simulink model "PreCondition"  (R2018b)
settings: Solver=FixedStepDiscrete  StartTime=0.0  StopTime=10.0  FixedStep=0.01  RelTol=1e-3
undefined symbols (not defined in the file or in its folder): EnergyMgLdShdRq1, HMI_2L_StMd10_Config_Val, HMI_2L_StMd11_Config_Val, HMI_2L_StMd12_Config_Val, HMI_2L_StMd13_Config_Val, HMI_2L_StMd14_Config_Val, HMI_2L_StMd15_Config_Val, HMI_2L_StMd16_Config_Val, HMI_2L_StMd17_Config_Val, HMI_2L_StMd18_Config_Val, HMI_2L_StMd19_Config_Val, HMI_2L_StMd1_Config_Val, HMI_2L_StMd20_Config_Val, HMI_2L_StMd21_Config_Val, HMI_2L_StMd22_Config_Val, HMI_2L_StMd23_Config_Val, HMI_2L_StMd24_Config_Val, HMI_2L_StMd25_Config_Val, HMI_2L_StMd26_Config_Val, HMI_2L_StMd27_Config_Val, HMI_2L_StMd28_Config_Val, HMI_2L_StMd29_Config_Val, HMI_2L_StMd2_Config_Val, HMI_2L_StMd30_Config_Val, HMI_2L_StMd31_Config_Val, HMI_2L_StMd32_Config_Val, HMI_2L_StMd3_Config_Val, HMI_2L_StMd4_Config_Val, HMI_2L_StMd5_Config_Val, HMI_2L_StMd6_Config_Val, HMI_2L_StMd7_Config_Val, HMI_2L_StMd8_Config_Val, HMI_2L_StMd9_Config_Val, HMI_2R_StMd10_Config_Val, HMI_2R_StMd11_Config_Val, HMI_2R_StMd12_Config_Val, HMI_2R_StMd13_Config_Val, HMI_2R_StMd14_Config_Val, HMI_2R_StMd15_Config_Val, HMI_2R_StMd16_Config_Val, HMI_2R_StMd17_Config_Val, HMI_2R_StMd18_Config_Val, HMI_2R_StMd19_Config_Val, HMI_2R_StMd1_Config_Val, HMI_2R_StMd20_Config_Val, HMI_2R_StMd21_Config_Val, HMI_2R_StMd22_Config_Val, HMI_2R_StMd23_Config_Val, HMI_2R_StMd24_Config_Val, HMI_2R_StMd25_Config_Val, HMI_2R_StMd26_Config_Val, HMI_2R_StMd27_Config_Val, HMI_2R_StMd28_Config_Val, HMI_2R_StMd29_Config_Val, HMI_2R_StMd2_Config_Val, HMI_2R_StMd30_Config_Val, HMI_2R_StMd31_Config_Val, HMI_2R_StMd32_Config_Val, HMI_2R_StMd3_Config_Val, HMI_2R_StMd4_Config_Val ... (+94)
(part 3 of 6)

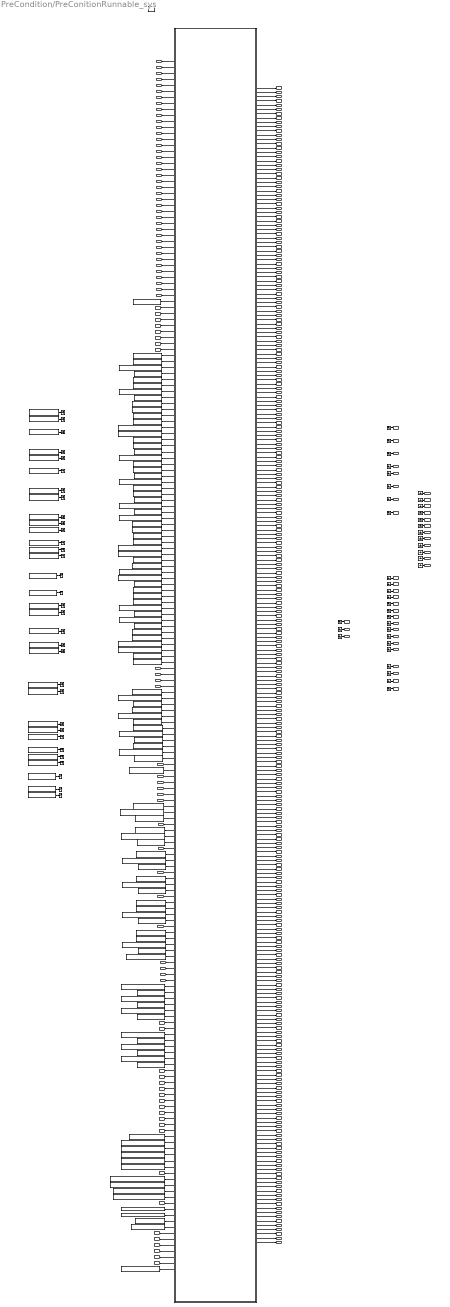
== system PreCondition/PreConitionRunnable_sys ==
  AbgDplyBckp_Val_read : Inport
  AbgDplyBckpV_Val_read : Inport  Port=2
  AcsEntryPosLrnd_Val_read : Inport  Port=3
  DrvStPosRclRspStat_Val_read : Inport  Port=4
  EnergyMgLdShdRq_Val_read : Inport  Port=5
  FamilyLtPosLrnd_Val_read : Inport  Port=6
  FamilyRtPosLrnd_Val_read : Inport  Port=7
  IfVeSMSeStNumConfig_Val_read : Inport  Port=8
  IntimacyLPosLrnd_Val_read : Inport  Port=9
  IntimacyRPosLrnd_Val_read : Inport  Port=10
  Is2LStSwAct_Val_read : Inport  Port=11
  Is2RStSwAct_Val_read : Inport  Port=12
  Is3LStSwAct_Val_read : Inport  Port=13
  Is3RStSwAct_Val_read : Inport  Port=14
  IsDrvStSwAct_Val_read : Inport  Port=15
  IsPasStSwAct_Val_read : Inport  Port=16
  LgrstCloseLtPosLrnd_Val_read : Inport  Port=17
  LgrstCloseRtPosLrnd_Val_read : Inport  Port=18
  LgrstOpenLtPosLrnd_Val_read : Inport  Port=19
  LgrstOpenRtPosLrnd_Val_read : Inport  Port=20
  LugLtPosLrnd_Val_read : Inport  Port=21
  LugRtPosLrnd_Val_read : Inport  Port=22
  LyingLtPosLrnd_Val_read : Inport  Port=23
  LyingRtPosLrnd_Val_read : Inport  Port=24
  MmryRclImpctDisRq_Val_read : Inport  Port=25
  AcsExitPosLrnd_Val_read : Inport  Port=26
  PassStPosRclRspStat_Val_read : Inport  Port=27
  VIPLtPosLrnd_Val_read : Inport  Port=28
  SecRwLtStChldLkReq_Val_read : Inport  Port=29
  SecRwLtStPosRclRspStat_Val_read : Inport  Port=30
  VIPRtPosLrnd_Val_read : Inport  Port=31
  SecRwRtStChldLkReq_Val_read : Inport  Port=32
  SecRwRtStPosRclRspStat_Val_read : Inport  Port=33
  SysPwrMd_Val_read : Inport  Port=34
  SysPwrMdV_Val_read : Inport  Port=35
  ThdRwCtStOccStatMSMSrc_Val_read : Inport  Port=36
  RcvyLtPosLrnd_Val_read : Inport  Port=37
  ThdRwLtStOccStatMSMSrc_Val_read : Inport  Port=38
  ThdRwLtStPosRclRspStat_Val_read : Inport  Port=39
  RcvyRtPosLrnd_Val_read : Inport  Port=40
  ThdRwRtStOccStatMSMSrc_Val_read : Inport  Port=41
  ThdRwRtStPosRclRspStat_Val_read : Inport  Port=42
  VehMovState_Val_read : Inport  Port=43
  VehSpdAvgDrvn_Val_read : Inport  Port=44
  VehSpdAvgDrvnV_Val_read : Inport  Port=45
  VeSignalLost2R_463_2L_Val_read : Inport  Port=46
  VeSignalLost3L_468_2L_Val_read : Inport  Port=47
  VeSignalLost3R_46C_2L_Val_read : Inport  Port=48
  VeSignalLostCODR_470_2L_Val_read : Inport  Port=49
  VeSignalLostDR_213_2L_Val_read : Inport  Port=50
  VeSignalLostFireWall_1D2_2L_Val_read : Inport  Port=51
  VeSignalLostSDM_195_2L_Val_read : Inport  Port=52
  VoltSts_Val_read : Inport  Port=53
  SecRwLtStFrwdBkwdPos_Val_read : Inport  Port=54
  SecRwLtStFrwdBkwdPosV_Val_read : Inport  Port=55
  SecRwRtStFrwdBkwdPos_Val_read : Inport  Port=56
  SecRwRtStFrwdBkwdPosV_Val_read : Inport  Port=57
  AcsEntry4s2LPosLrnd_Val_read : Inport  Port=58
  AcsEntry4s2RPosLrnd_Val_read : Inport  Port=59
  AcsEntryAll4sBwdPosLrnd_Val_read : Inport  Port=60
  AcsEntryAll4sFwdPosLrnd_Val_read : Inport  Port=61
  AcsExit4s2LPosLrnd_Val_read : Inport  Port=62
  AcsExit4s2RPosLrnd_Val_read : Inport  Port=63
  IfVeSMSbPassReclinerPosLrnd_Val_read : Inport  Port=64
  IfVeSMSbunfold3LPosLrnd_Val_read : Inport  Port=65
  IfVeSMSbunfold3RPosLrnd_Val_read : Inport  Port=66
  NotCoDrvStOccStatBDFSrc_Val_read : Inport  Port=67
  IfVeSMSbVIPLtOutPosLrnd_Val_read : Inport  Port=68
  IfVeSMSbVIPRtOutPosLrnd_Val_read : Inport  Port=69
  IfVeSMSuThdRwLtStCshnFldUpwdDnwdPos_Val_read : Inport  Port=70
  IfVeSMSuThdRwLtStCshnFldUpwdDnwdPosV_Val_read : Inport  Port=71
  IfVeSMSuThdRwRtStCshnFldUpwdDnwdPos_Val_read : Inport  Port=72
  IfVeSMSuThdRwRtStCshnFldUpwdDnwdPosV_Val_read : Inport  Port=73
  ThdRwLtStChldLkReq_Val_read : Inport  Port=74
  NotSecRowLeStOccStatBDFSrc_Val_read : Inport  Port=75
  NotSecRowRtStOccStatBDFSrc_Val_read : Inport  Port=76
  IfVeSMSbSecRwLtStBkReclnUpwdDnwdPosV_Val_read : Inport  Port=77
  IfVeSMSbSecRwRtStBkReclnUpwdDnwdPosV_Val_read : Inport  Port=78
  IfVeSMSuSecRwLtStBkReclnUpwdDnwdPos_Val_read : Inport  Port=79
  IfVeSMSuSecRwRtStBkReclnUpwdDnwdPos_Val_read : Inport  Port=80
  IfVeSMSbPasReclinerPosAvail_Val_read : Inport  Port=81
  WholeVehMemPosLrnd_Val_read : Inport  Port=82
  Md61PassStBkReclnTrgtPos_Val_read : Inport  Port=83
  Md61ThdRwLtStCshnFldUpwdDnwdTrgtPos_Val_read : Inport  Port=84
  Md61ThdRwRtStCshnFldUpwdDnwdTrgtPos_Val_read : Inport  Port=85
  Md62PassStBkReclnTrgtPos_Val_read : Inport  Port=86
  Md62ThdRwLtStCshnFldUpwdDnwdTrgtPos_Val_read : Inport  Port=87
  Md62ThdRwRtStCshnFldUpwdDnwdTrgtPos_Val_read : Inport  Port=88
  function : TriggerPort  TriggerType=function-call  VariantControl=(inherit)  SampleTimeType=periodic  SampleTime=-1
  Ground_{36,40,43,47,55,57,60,62,64,66..67,69,71,73,83..94,99..110,120} (39 alike) : Ground
  PA_HMI_2L_StMd10_Config_Val : Constant  Value=HMI_2L_StMd10_Config_Val
  PA_HMI_2L_StMd11_Config_Val : Constant  Value=HMI_2L_StMd11_Config_Val
  PA_HMI_2L_StMd12_Config_Val : Constant  Value=HMI_2L_StMd12_Config_Val
  PA_HMI_2L_StMd13_Config_Val : Constant  Value=HMI_2L_StMd13_Config_Val
  PA_HMI_2L_StMd14_Config_Val : Constant  Value=HMI_2L_StMd14_Config_Val
  PA_HMI_2L_StMd15_Config_Val : Constant  Value=HMI_2L_StMd15_Config_Val
  PA_HMI_2L_StMd16_Config_Val : Constant  Value=HMI_2L_StMd16_Config_Val
  PA_HMI_2L_StMd17_Config_Val : Constant  Value=HMI_2L_StMd17_Config_Val
  PA_HMI_2L_StMd18_Config_Val : Constant  Value=HMI_2L_StMd18_Config_Val
  PA_HMI_2L_StMd19_Config_Val : Constant  Value=HMI_2L_StMd19_Config_Val
  PA_HMI_2L_StMd1_Config_Val : Constant  Value=HMI_2L_StMd1_Config_Val
  PA_HMI_2L_StMd20_Config_Val : Constant  Value=HMI_2L_StMd20_Config_Val
  PA_HMI_2L_StMd21_Config_Val : Constant  Value=HMI_2L_StMd21_Config_Val
  PA_HMI_2L_StMd22_Config_Val : Constant  Value=HMI_2L_StMd22_Config_Val
  PA_HMI_2L_StMd23_Config_Val : Constant  Value=HMI_2L_StMd23_Config_Val
  PA_HMI_2L_StMd24_Config_Val : Constant  Value=HMI_2L_StMd24_Config_Val
  PA_HMI_2L_StMd25_Config_Val : Constant  Value=HMI_2L_StMd25_Config_Val
  PA_HMI_2L_StMd26_Config_Val : Constant  Value=HMI_2L_StMd26_Config_Val
  PA_HMI_2L_StMd27_Config_Val : Constant  Value=HMI_2L_StMd27_Config_Val
  PA_HMI_2L_StMd28_Config_Val : Constant  Value=HMI_2L_StMd28_Config_Val
  PA_HMI_2L_StMd29_Config_Val : Constant  Value=HMI_2L_StMd29_Config_Val
  PA_HMI_2L_StMd2_Config_Val : Constant  Value=HMI_2L_StMd2_Config_Val
  PA_HMI_2L_StMd30_Config_Val : Constant  Value=HMI_2L_StMd30_Config_Val
  PA_HMI_2L_StMd31_Config_Val : Constant  Value=HMI_2L_StMd31_Config_Val
  PA_HMI_2L_StMd32_Config_Val : Constant  Value=HMI_2L_StMd32_Config_Val
  PA_HMI_2L_StMd3_Config_Val : Constant  Value=HMI_2L_StMd3_Config_Val
  PA_HMI_2L_StMd4_Config_Val : Constant  Value=HMI_2L_StMd4_Config_Val
  PA_HMI_2L_StMd5_Config_Val : Constant  Value=HMI_2L_StMd5_Config_Val
  PA_HMI_2L_StMd6_Config_Val : Constant  Value=HMI_2L_StMd6_Config_Val
  PA_HMI_2L_StMd7_Config_Val : Constant  Value=HMI_2L_StMd7_Config_Val
  PA_HMI_2L_StMd8_Config_Val : Constant  Value=HMI_2L_StMd8_Config_Val
  PA_HMI_2L_StMd9_Config_Val : Constant  Value=HMI_2L_StMd9_Config_Val
  PA_HMI_2R_StMd10_Config_Val : Constant  Value=HMI_2R_StMd10_Config_Val
  PA_HMI_2R_StMd11_Config_Val : Constant  Value=HMI_2R_StMd11_Config_Val
  PA_HMI_2R_StMd12_Config_Val : Constant  Value=HMI_2R_StMd12_Config_Val
  PA_HMI_2R_StMd13_Config_Val : Constant  Value=HMI_2R_StMd13_Config_Val
  PA_HMI_2R_StMd14_Config_Val : Constant  Value=HMI_2R_StMd14_Config_Val
  PA_HMI_2R_StMd15_Config_Val : Constant  Value=HMI_2R_StMd15_Config_Val
  PA_HMI_2R_StMd16_Config_Val : Constant  Value=HMI_2R_StMd16_Config_Val
  PA_HMI_2R_StMd17_Config_Val : Constant  Value=HMI_2R_StMd17_Config_Val
  PA_HMI_2R_StMd18_Config_Val : Constant  Value=HMI_2R_StMd18_Config_Val
  PA_HMI_2R_StMd19_Config_Val : Constant  Value=HMI_2R_StMd19_Config_Val
  PA_HMI_2R_StMd1_Config_Val : Constant  Value=HMI_2R_StMd1_Config_Val
  PA_HMI_2R_StMd20_Config_Val : Constant  Value=HMI_2R_StMd20_Config_Val
  PA_HMI_2R_StMd21_Config_Val : Constant  Value=HMI_2R_StMd21_Config_Val
  PA_HMI_2R_StMd22_Config_Val : Constant  Value=HMI_2R_StMd22_Config_Val
  PA_HMI_2R_StMd23_Config_Val : Constant  Value=HMI_2R_StMd23_Config_Val
  PA_HMI_2R_StMd24_Config_Val : Constant  Value=HMI_2R_StMd24_Config_Val
  PA_HMI_2R_StMd25_Config_Val : Constant  Value=HMI_2R_StMd25_Config_Val
  PA_HMI_2R_StMd26_Config_Val : Constant  Value=HMI_2R_StMd26_Config_Val
  PA_HMI_2R_StMd27_Config_Val : Constant  Value=HMI_2R_StMd27_Config_Val
  PA_HMI_2R_StMd28_Config_Val : Constant  Value=HMI_2R_StMd28_Config_Val
  PA_HMI_2R_StMd29_Config_Val : Constant  Value=HMI_2R_StMd29_Config_Val
  PA_HMI_2R_StMd2_Config_Val : Constant  Value=HMI_2R_StMd2_Config_Val
  PA_HMI_2R_StMd30_Config_Val : Constant  Value=HMI_2R_StMd30_Config_Val
  PA_HMI_2R_StMd31_Config_Val : Constant  Value=HMI_2R_StMd31_Config_Val
  PA_HMI_2R_StMd32_Config_Val : Constant  Value=HMI_2R_StMd32_Config_Val
  PA_HMI_2R_StMd3_Config_Val : Constant  Value=HMI_2R_StMd3_Config_Val
  PA_HMI_2R_StMd4_Config_Val : Constant  Value=HMI_2R_StMd4_Config_Val
  PA_HMI_2R_StMd5_Config_Val : Constant  Value=HMI_2R_StMd5_Config_Val
  PA_HMI_2R_StMd6_Config_Val : Constant  Value=HMI_2R_StMd6_Config_Val
  PA_HMI_2R_StMd7_Config_Val : Constant  Value=HMI_2R_StMd7_Config_Val
  PA_HMI_2R_StMd8_Config_Val : Constant  Value=HMI_2R_StMd8_Config_Val
  PA_HMI_2R_StMd9_Config_Val : Constant  Value=HMI_2R_StMd9_Config_Val
  PA_IfKeSMSbSeatMovFrwdBkwdEnable_Val : Constant  Value=IfKeSMSbSeatMovFrwdBkwdEnable_Val
  PA_KeSMSLegrstDisFwdBkwdPos_Val : Constant  Value=KeSMSLegrstDisFwdBkwdPos_Val
  PA_KeSMSbRoofSWEnable_Val : Constant  Value=KeSMSbRoofSWEnable_Val
  PA_KeSMSuSecRwStBackPosDelta_Val : Constant  Value=KeSMSuSecRwStBackPosDelta_Val
  PA_KeSMSuThrdRwCushFoldPosDelta_Val : Constant  Value=KeSMSuThrdRwCushFoldPosDelta_Val
  PA_KeSMSuThrdRwCushFoldPosThreshold_Val : Constant  Value=KeSMSuThrdRwCushFoldPosThreshold_Val
  PA_KeSMSwAcsMd32SecRwLtStBkReclnUpwdDnwdPos1_Val : Constant  Value=KeSMSwAcsMd32SecRwLtStBkReclnUpwdDnwdPos1_Val
  PA_KeSMSwAcsMd53SecRwRtStBkReclnUpwdDnwdPos1_Val : Constant  Value=KeSMSwAcsMd53SecRwRtStBkReclnUpwdDnwdPos1_Val
  PA_KeSMSwAcsMd8SecRwLtStBkReclnUpwdDnwdPos_Val : Constant  Value=KeSMSwAcsMd8SecRwLtStBkReclnUpwdDnwdPos_Val
  PA_KeSMSwAcsMd9SecRwRtStBkReclnUpwdDnwdPos_Val : Constant  Value=KeSMSwAcsMd9SecRwRtStBkReclnUpwdDnwdPos_Val
  PA_KeSMSwSeatBkLimitPosDelt_Val : Constant  Value=KeSMSwSeatBkLimitPosDelt_Val
  PA_KeSMSwSeatBkLimitPos_Val : Constant  Value=KeSMSwSeatBkLimitPos_Val
  PA_StPassCmprtMdCtrl_Md10_VCUConfig_Val : Constant  Value=StPassCmprtMdCtrl_Md10_VCUConfig_Val
  PA_StPassCmprtMdCtrl_Md11_VCUConfig_Val : Constant  Value=StPassCmprtMdCtrl_Md11_VCUConfig_Val
  PA_StPassCmprtMdCtrl_Md12_VCUConfig_Val : Constant  Value=StPassCmprtMdCtrl_Md12_VCUConfig_Val
  PA_StPassCmprtMdCtrl_Md13_VCUConfig_Val : Constant  Value=StPassCmprtMdCtrl_Md13_VCUConfig_Val
  PA_StPassCmprtMdCtrl_Md14_VCUConfig_Val : Constant  Value=StPassCmprtMdCtrl_Md14_VCUConfig_Val
  PA_StPassCmprtMdCtrl_Md15_VCUConfig_Val : Constant  Value=StPassCmprtMdCtrl_Md15_VCUConfig_Val
  PA_StPassCmprtMdCtrl_Md16_VCUConfig_Val : Constant  Value=StPassCmprtMdCtrl_Md16_VCUConfig_Val
  PA_StPassCmprtMdCtrl_Md17_VCUConfig_Val : Constant  Value=StPassCmprtMdCtrl_Md17_VCUConfig_Val
  PA_StPassCmprtMdCtrl_Md18_VCUConfig_Val : Constant  Value=StPassCmprtMdCtrl_Md18_VCUConfig_Val
  PA_StPassCmprtMdCtrl_Md19_VCUConfig_Val : Constant  Value=StPassCmprtMdCtrl_Md19_VCUConfig_Val
  PA_StPassCmprtMdCtrl_Md1_VCUConfig_Val : Constant  Value=StPassCmprtMdCtrl_Md1_VCUConfig_Val
  PA_StPassCmprtMdCtrl_Md20_VCUConfig_Val : Constant  Value=StPassCmprtMdCtrl_Md20_VCUConfig_Val
  PA_StPassCmprtMdCtrl_Md21_VCUConfig_Val : Constant  Value=StPassCmprtMdCtrl_Md21_VCUConfig_Val
  PA_StPassCmprtMdCtrl_Md22_VCUConfig_Val : Constant  Value=StPassCmprtMdCtrl_Md22_VCUConfig_Val
  PA_StPassCmprtMdCtrl_Md23_VCUConfig_Val : Constant  Value=StPassCmprtMdCtrl_Md23_VCUConfig_Val
  PA_StPassCmprtMdCtrl_Md24_VCUConfig_Val : Constant  Value=StPassCmprtMdCtrl_Md24_VCUConfig_Val
  PA_StPassCmprtMdCtrl_Md25_VCUConfig_Val : Constant  Value=StPassCmprtMdCtrl_Md25_VCUConfig_Val
  PA_StPassCmprtMdCtrl_Md26_VCUConfig_Val : Constant  Value=StPassCmprtMdCtrl_Md26_VCUConfig_Val
  PA_StPassCmprtMdCtrl_Md27_VCUConfig_Val : Constant  Value=StPassCmprtMdCtrl_Md27_VCUConfig_Val
  PA_StPassCmprtMdCtrl_Md28_VCUConfig_Val : Constant  Value=StPassCmprtMdCtrl_Md28_VCUConfig_Val
  PA_StPassCmprtMdCtrl_Md29_VCUConfig_Val : Constant  Value=StPassCmprtMdCtrl_Md29_VCUConfig_Val
  PA_StPassCmprtMdCtrl_Md2_VCUConfig_Val : Constant  Value=StPassCmprtMdCtrl_Md2_VCUConfig_Val
  PA_StPassCmprtMdCtrl_Md30_VCUConfig_Val : Constant  Value=StPassCmprtMdCtrl_Md30_VCUConfig_Val
  PA_StPassCmprtMdCtrl_Md31_VCUConfig_Val : Constant  Value=StPassCmprtMdCtrl_Md31_VCUConfig_Val
  PA_StPassCmprtMdCtrl_Md32_VCUConfig_Val : Constant  Value=StPassCmprtMdCtrl_Md32_VCUConfig_Val
  PA_StPassCmprtMdCtrl_Md3_VCUConfig_Val : Constant  Value=StPassCmprtMdCtrl_Md3_VCUConfig_Val
  PA_StPassCmprtMdCtrl_Md4_VCUConfig_Val : Constant  Value=StPassCmprtMdCtrl_Md4_VCUConfig_Val
  PA_StPassCmprtMdCtrl_Md53_VCUConfig_Val : Constant  Value=StPassCmprtMdCtrl_Md53_VCUConfig_Val
  PA_StPassCmprtMdCtrl_Md56_VCUConfig_Val : Constant  Value=StPassCmprtMdCtrl_Md56_VCUConfig_Val
  PA_StPassCmprtMdCtrl_Md57_VCUConfig_Val : Constant  Value=StPassCmprtMdCtrl_Md57_VCUConfig_Val
  PA_StPassCmprtMdCtrl_Md58_VCUConfig_Val : Constant  Value=StPassCmprtMdCtrl_Md58_VCUConfig_Val
  PA_StPassCmprtMdCtrl_Md5_VCUConfig_Val : Constant  Value=StPassCmprtMdCtrl_Md5_VCUConfig_Val
  PA_StPassCmprtMdCtrl_Md61_VCUConfig_Val : Constant  Value=StPassCmprtMdCtrl_Md61_VCUConfig_Val
  PA_StPassCmprtMdCtrl_Md62_VCUConfig_Val : Constant  Value=StPassCmprtMdCtrl_Md62_VCUConfig_Val
  PA_StPassCmprtMdCtrl_Md6_VCUConfig_Val : Constant  Value=StPassCmprtMdCtrl_Md6_VCUConfig_Val
  PA_StPassCmprtMdCtrl_Md7_VCUConfig_Val : Constant  Value=StPassCmprtMdCtrl_Md7_VCUConfig_Val
  PA_StPassCmprtMdCtrl_Md8_VCUConfig_Val : Constant  Value=StPassCmprtMdCtrl_Md8_VCUConfig_Val
  PA_StPassCmprtMdCtrl_Md9_VCUConfig_Val : Constant  Value=StPassCmprtMdCtrl_Md9_VCUConfig_Val
  PA_StSrv_StMd10_Config_Val : Constant  Value=StSrv_StMd10_Config_Val
  PA_StSrv_StMd11_Config_Val : Constant  Value=StSrv_StMd11_Config_Val
  PA_StSrv_StMd12_Config_Val : Constant  Value=StSrv_StMd12_Config_Val
  PA_StSrv_StMd13_Config_Val : Constant  Value=StSrv_StMd13_Config_Val
  PA_StSrv_StMd14_Config_Val : Constant  Value=StSrv_StMd14_Config_Val
  PA_StSrv_StMd15_Config_Val : Constant  Value=StSrv_StMd15_Config_Val
  PA_StSrv_StMd16_Config_Val : Constant  Value=StSrv_StMd16_Config_Val
  PA_StSrv_StMd17_Config_Val : Constant  Value=StSrv_StMd17_Config_Val
  PA_StSrv_StMd18_Config_Val : Constant  Value=StSrv_StMd18_Config_Val
  PA_StSrv_StMd19_Config_Val : Constant  Value=StSrv_StMd19_Config_Val
  PA_StSrv_StMd1_Config_Val : Constant  Value=StSrv_StMd1_Config_Val
  PA_StSrv_StMd20_Config_Val : Constant  Value=StSrv_StMd20_Config_Val
  PA_StSrv_StMd21_Config_Val : Constant  Value=StSrv_StMd21_Config_Val
  PA_StSrv_StMd22_Config_Val : Constant  Value=StSrv_StMd22_Config_Val
  PA_StSrv_StMd23_Config_Val : Constant  Value=StSrv_StMd23_Config_Val
  PA_StSrv_StMd24_Config_Val : Constant  Value=StSrv_StMd24_Config_Val
  PA_StSrv_StMd25_Config_Val : Constant  Value=StSrv_StMd25_Config_Val
  PA_StSrv_StMd26_Config_Val : Constant  Value=StSrv_StMd26_Config_Val
  PA_StSrv_StMd27_Config_Val : Constant  Value=StSrv_StMd27_Config_Val
  PA_StSrv_StMd28_Config_Val : Constant  Value=StSrv_StMd28_Config_Val
  PA_StSrv_StMd29_Config_Val : Constant  Value=StSrv_StMd29_Config_Val
  PA_StSrv_StMd2_Config_Val : Constant  Value=StSrv_StMd2_Config_Val
  PA_StSrv_StMd30_Config_Val : Constant  Value=StSrv_StMd30_Config_Val
  PA_StSrv_StMd31_Config_Val : Constant  Value=StSrv_StMd31_Config_Val
  PA_StSrv_StMd32_Config_Val : Constant  Value=StSrv_StMd32_Config_Val
  PA_StSrv_StMd3_Config_Val : Constant  Value=StSrv_StMd3_Config_Val
  PA_StSrv_StMd4_Config_Val : Constant  Value=StSrv_StMd4_Config_Val
  PA_StSrv_StMd5_Config_Val : Constant  Value=StSrv_StMd5_Config_Val
  PA_StSrv_StMd6_Config_Val : Constant  Value=StSrv_StMd6_Config_Val
  PA_StSrv_StMd7_Config_Val : Constant  Value=StSrv_StMd7_Config_Val
  PA_StSrv_StMd8_Config_Val : Constant  Value=StSrv_StMd8_Config_Val
  PA_StSrv_StMd9_Config_Val : Constant  Value=StSrv_StMd9_Config_Val
  Subsystem3 : Subsystem
  Terminator_{56..57,59,62..63,65,68..69,72..74,76..78,82,85..87,90,92..93,98..99,104..106,108..110,113,115..116} (32 alike) : Terminator
  AcsMdEntyAvl_Val_write : Outport
  AcsMdExtAvl_Val_write : Outport  Port=2
  CommCond_Val_write : Outport  Port=3
  CommExitCond_Val_write : Outport  Port=4
  CommExitCondwithSpeed_Val_write : Outport  Port=5
  DiagAbgDly_Val_write : Outport  Port=6
  DiagVehMovState_Val_write : Outport  Port=7
  DiagVehSpdAvgDrvn_Val_write : Outport  Port=8
  FamilyMdLtAvl_Val_write : Outport  Port=9
  FamilyMdRtAvl_Val_write : Outport  Port=10
  HMIMd10Avl_2L_Val_write : Outport  Port=11
  HMIMd10Avl_2R_Val_write : Outport  Port=12
  HMIMd10Cfg_2L_Val_write : Outport  Port=13
  HMIMd10Cfg_2R_Val_write : Outport  Port=14
  HMIMd11Avl_2L_Val_write : Outport  Port=15
  HMIMd11Avl_2R_Val_write : Outport  Port=16
  HMIMd11Cfg_2L_Val_write : Outport  Port=17
  HMIMd11Cfg_2R_Val_write : Outport  Port=18
  HMIMd12Avl_2L_Val_write : Outport  Port=19
  HMIMd12Avl_2R_Val_write : Outport  Port=20
  HMIMd12Cfg_2L_Val_write : Outport  Port=21
  HMIMd12Cfg_2R_Val_write : Outport  Port=22
  HMIMd13Avl_2L_Val_write : Outport  Port=23
  HMIMd13Avl_2R_Val_write : Outport  Port=24
  HMIMd13Cfg_2L_Val_write : Outport  Port=25
  HMIMd13Cfg_2R_Val_write : Outport  Port=26
  HMIMd14Avl_2L_Val_write : Outport  Port=27
  HMIMd14Avl_2R_Val_write : Outport  Port=28
  HMIMd14Cfg_2L_Val_write : Outport  Port=29
  HMIMd14Cfg_2R_Val_write : Outport  Port=30
  HMIMd15Avl_2L_Val_write : Outport  Port=31
  HMIMd15Avl_2R_Val_write : Outport  Port=32
  HMIMd15Cfg_2L_Val_write : Outport  Port=33
  HMIMd15Cfg_2R_Val_write : Outport  Port=34
  HMIMd16Avl_2L_Val_write : Outport  Port=35
  HMIMd16Avl_2R_Val_write : Outport  Port=36
      settings: EnsureOutportIsVirtual=on
  HMIMd16Cfg_2L_Val_write : Outport  Port=37
  HMIMd16Cfg_2R_Val_write : Outport  Port=38
  HMIMd17Avl_2L_Val_write : Outport  Port=39
  HMIMd17Avl_2R_Val_write : Outport  Port=40
      settings: EnsureOutportIsVirtual=on
  HMIMd17Cfg_2L_Val_write : Outport  Port=41
  HMIMd17Cfg_2R_Val_write : Outport  Port=42
  HMIMd18Avl_2L_Val_write : Outport  Port=43
      settings: EnsureOutportIsVirtual=on
  HMIMd18Avl_2R_Val_write : Outport  Port=44
  HMIMd18Cfg_2L_Val_write : Outport  Port=45
  HMIMd18Cfg_2R_Val_write : Outport  Port=46
  HMIMd19Avl_2L_Val_write : Outport  Port=47
      settings: EnsureOutportIsVirtual=on
  HMIMd19Avl_2R_Val_write : Outport  Port=48
  HMIMd19Cfg_2L_Val_write : Outport  Port=49
  HMIMd19Cfg_2R_Val_write : Outport  Port=50
  HMIMd1Avl_2L_Val_write : Outport  Port=51
  HMIMd1Avl_2R_Val_write : Outport  Port=52
  HMIMd1Cfg_2L_Val_write : Outport  Port=53
  HMIMd1Cfg_2R_Val_write : Outport  Port=54
  HMIMd20Avl_2L_Val_write : Outport  Port=55
      settings: EnsureOutportIsVirtual=on
  HMIMd20Avl_2R_Val_write : Outport  Port=56
  HMIMd20Cfg_2L_Val_write : Outport  Port=57
      settings: EnsureOutportIsVirtual=on
  HMIMd20Cfg_2R_Val_write : Outport  Port=58
  HMIMd21Avl_2L_Val_write : Outport  Port=59
  HMIMd21Avl_2R_Val_write : Outport  Port=60
      settings: EnsureOutportIsVirtual=on
  HMIMd21Cfg_2L_Val_write : Outport  Port=61
  HMIMd21Cfg_2R_Val_write : Outport  Port=62
      settings: EnsureOutportIsVirtual=on
  HMIMd22Avl_2L_Val_write : Outport  Port=63
  HMIMd22Avl_2R_Val_write : Outport  Port=64
      settings: EnsureOutportIsVirtual=on
  HMIMd22Cfg_2L_Val_write : Outport  Port=65
  HMIMd22Cfg_2R_Val_write : Outport  Port=66
      settings: EnsureOutportIsVirtual=on
  HMIMd23Avl_2L_Val_write : Outport  Port=67
      settings: EnsureOutportIsVirtual=on
  HMIMd23Avl_2R_Val_write : Outport  Port=68
  HMIMd23Cfg_2L_Val_write : Outport  Port=69
      settings: EnsureOutportIsVirtual=on
  HMIMd23Cfg_2R_Val_write : Outport  Port=70
  HMIMd24Avl_2L_Val_write : Outport  Port=71
      settings: EnsureOutportIsVirtual=on
  HMIMd24Avl_2R_Val_write : Outport  Port=72
  HMIMd24Cfg_2L_Val_write : Outport  Port=73
      settings: EnsureOutportIsVirtual=on
  HMIMd24Cfg_2R_Val_write : Outport  Port=74
  HMIMd25Avl_2L_Val_write : Outport  Port=75
  HMIMd25Avl_2R_Val_write : Outport  Port=76
  HMIMd25Cfg_2L_Val_write : Outport  Port=77
  HMIMd25Cfg_2R_Val_write : Outport  Port=78
  HMIMd26Avl_2L_Val_write : Outport  Port=79
  HMIMd26Avl_2R_Val_write : Outport  Port=80
  HMIMd26Cfg_2L_Val_write : Outport  Port=81
  HMIMd26Cfg_2R_Val_write : Outport  Port=82
  HMIMd27Avl_2L_Val_write : Outport  Port=83
      settings: EnsureOutportIsVirtual=on
  HMIMd27Avl_2R_Val_write : Outport  Port=84
      settings: EnsureOutportIsVirtual=on
  HMIMd27Cfg_2L_Val_write : Outport  Port=85
      settings: EnsureOutportIsVirtual=on
  HMIMd27Cfg_2R_Val_write : Outport  Port=86
      settings: EnsureOutportIsVirtual=on
  HMIMd28Avl_2L_Val_write : Outport  Port=87
      settings: EnsureOutportIsVirtual=on
  HMIMd28Avl_2R_Val_write : Outport  Port=88
      settings: EnsureOutportIsVirtual=on
  HMIMd28Cfg_2L_Val_write : Outport  Port=89
      settings: EnsureOutportIsVirtual=on
  HMIMd28Cfg_2R_Val_write : Outport  Port=90
      settings: EnsureOutportIsVirtual=on
  HMIMd29Avl_2L_Val_write : Outport  Port=91
      settings: EnsureOutportIsVirtual=on
  HMIMd29Avl_2R_Val_write : Outport  Port=92
      settings: EnsureOutportIsVirtual=on
  HMIMd29Cfg_2L_Val_write : Outport  Port=93
      settings: EnsureOutportIsVirtual=on
  HMIMd29Cfg_2R_Val_write : Outport  Port=94
      settings: EnsureOutportIsVirtual=on
  HMIMd2Avl_2L_Val_write : Outport  Port=95
  HMIMd2Avl_2R_Val_write : Outport  Port=96
  HMIMd2Cfg_2L_Val_write : Outport  Port=97
  HMIMd2Cfg_2R_Val_write : Outport  Port=98
  HMIMd30Avl_2L_Val_write : Outport  Port=99
      settings: EnsureOutportIsVirtual=on
  HMIMd30Avl_2R_Val_write : Outport  Port=100
      settings: EnsureOutportIsVirtual=on
  HMIMd30Cfg_2L_Val_write : Outport  Port=101
      settings: EnsureOutportIsVirtual=on
  HMIMd30Cfg_2R_Val_write : Outport  Port=102
      settings: EnsureOutportIsVirtual=on
  HMIMd31Avl_2L_Val_write : Outport  Port=103
      settings: EnsureOutportIsVirtual=on
  HMIMd31Avl_2R_Val_write : Outport  Port=104
      settings: EnsureOutportIsVirtual=on
  HMIMd31Cfg_2L_Val_write : Outport  Port=105
      settings: EnsureOutportIsVirtual=on
  HMIMd31Cfg_2R_Val_write : Outport  Port=106
      settings: EnsureOutportIsVirtual=on
  HMIMd32Avl_2L_Val_write : Outport  Port=107
      settings: EnsureOutportIsVirtual=on
  HMIMd32Avl_2R_Val_write : Outport  Port=108
      settings: EnsureOutportIsVirtual=on
  HMIMd32Cfg_2L_Val_write : Outport  Port=109
      settings: EnsureOutportIsVirtual=on
  HMIMd32Cfg_2R_Val_write : Outport  Port=110
      settings: EnsureOutportIsVirtual=on
  HMIMd3Avl_2L_Val_write : Outport  Port=111
  HMIMd3Avl_2R_Val_write : Outport  Port=112
  HMIMd3Cfg_2L_Val_write : Outport  Port=113
  HMIMd3Cfg_2R_Val_write : Outport  Port=114
  HMIMd4Avl_2L_Val_write : Outport  Port=115
  HMIMd4Avl_2R_Val_write : Outport  Port=116
  HMIMd4Cfg_2L_Val_write : Outport  Port=117
  HMIMd4Cfg_2R_Val_write : Outport  Port=118
  HMIMd5Avl_2L_Val_write : Outport  Port=119
  HMIMd5Avl_2R_Val_write : Outport  Port=120
      settings: EnsureOutportIsVirtual=on
  HMIMd5Cfg_2L_Val_write : Outport  Port=121
  HMIMd5Cfg_2R_Val_write : Outport  Port=122
  HMIMd6Avl_2L_Val_write : Outport  Port=123
  HMIMd6Avl_2R_Val_write : Outport  Port=124
  HMIMd6Cfg_2L_Val_write : Outport  Port=125
  HMIMd6Cfg_2R_Val_write : Outport  Port=126
  HMIMd7Avl_2L_Val_write : Outport  Port=127
  HMIMd7Avl_2R_Val_write : Outport  Port=128
  HMIMd7Cfg_2L_Val_write : Outport  Port=129
  HMIMd7Cfg_2R_Val_write : Outport  Port=130
  HMIMd8Avl_2L_Val_write : Outport  Port=131
  HMIMd8Avl_2R_Val_write : Outport  Port=132
  HMIMd8Cfg_2L_Val_write : Outport  Port=133
  HMIMd8Cfg_2R_Val_write : Outport  Port=134
  HMIMd9Avl_2L_Val_write : Outport  Port=135
  HMIMd9Avl_2R_Val_write : Outport  Port=136
  HMIMd9Cfg_2L_Val_write : Outport  Port=137
  HMIMd9Cfg_2R_Val_write : Outport  Port=138
  IntimacyLMdAvl_Val_write : Outport  Port=139
  IntimacyRMdAvl_Val_write : Outport  Port=140
  LgrstCloseLtMdAvl_Val_write : Outport  Port=141
  LgrstCloseRtMdAvl_Val_write : Outport  Port=142
  LgrstOpenLtMdAvl_Val_write : Outport  Port=143
  LgrstOpenRtMdAvl_Val_write : Outport  Port=144
  LugMdLtAvl_Val_write : Outport  Port=145
  LugMdRtAvl_Val_write : Outport  Port=146
  LyingMdLtAvl_Val_write : Outport  Port=147
  LyingMdRtAvl_Val_write : Outport  Port=148
  PwrMdChked_Val_write : Outport  Port=149
  RcvyMdLtAvl_Val_write : Outport  Port=150
  RcvyMdRtAvl_Val_write : Outport  Port=151
  StPassCmprtMdCtrl_Md1_VCUAvl_Val_write : Outport  Port=152
  StPassCmprtMdCtrl_Md1_VCUCfg_Val_write : Outport  Port=153
  StPassCmprtMdCtrl_Md10_VCUAvl_Val_write : Outport  Port=154
  StPassCmprtMdCtrl_Md10_VCUCfg_Val_write : Outport  Port=155
  StPassCmprtMdCtrl_Md11_VCUAvl_Val_write : Outport  Port=156
  StPassCmprtMdCtrl_Md11_VCUCfg_Val_write : Outport  Port=157
  StPassCmprtMdCtrl_Md12_VCUAvl_Val_write : Outport  Port=158
  StPassCmprtMdCtrl_Md12_VCUCfg_Val_write : Outport  Port=159
  StPassCmprtMdCtrl_Md13_VCUAvl_Val_write : Outport  Port=160
  StPassCmprtMdCtrl_Md13_VCUCfg_Val_write : Outport  Port=161
  StPassCmprtMdCtrl_Md14_VCUAvl_Val_write : Outport  Port=162
  StPassCmprtMdCtrl_Md14_VCUCfg_Val_write : Outport  Port=163
  StPassCmprtMdCtrl_Md15_VCUAvl_Val_write : Outport  Port=164
  StPassCmprtMdCtrl_Md15_VCUCfg_Val_write : Outport  Port=165
  StPassCmprtMdCtrl_Md16_VCUAvl_Val_write : Outport  Port=166
  StPassCmprtMdCtrl_Md16_VCUCfg_Val_write : Outport  Port=167
  StPassCmprtMdCtrl_Md17_VCUAvl_Val_write : Outport  Port=168
  StPassCmprtMdCtrl_Md17_VCUCfg_Val_write : Outport  Port=169
  StPassCmprtMdCtrl_Md18_VCUAvl_Val_write : Outport  Port=170
  StPassCmprtMdCtrl_Md18_VCUCfg_Val_write : Outport  Port=171
  StPassCmprtMdCtrl_Md19_VCUAvl_Val_write : Outport  Port=172
  StPassCmprtMdCtrl_Md19_VCUCfg_Val_write : Outport  Port=173
  StPassCmprtMdCtrl_Md2_VCUAvl_Val_write : Outport  Port=174
  StPassCmprtMdCtrl_Md2_VCUCfg_Val_write : Outport  Port=175
  StPassCmprtMdCtrl_Md20_VCUAvl_Val_write : Outport  Port=176
  StPassCmprtMdCtrl_Md20_VCUCfg_Val_write : Outport  Port=177
  StPassCmprtMdCtrl_Md21_VCUAvl_Val_write : Outport  Port=178
  StPassCmprtMdCtrl_Md21_VCUCfg_Val_write : Outport  Port=179
  StPassCmprtMdCtrl_Md22_VCUAvl_Val_write : Outport  Port=180
  StPassCmprtMdCtrl_Md22_VCUCfg_Val_write : Outport  Port=181
  StPassCmprtMdCtrl_Md23_VCUAvl_Val_write : Outport  Port=182
  StPassCmprtMdCtrl_Md23_VCUCfg_Val_write : Outport  Port=183
  StPassCmprtMdCtrl_Md24_VCUAvl_Val_write : Outport  Port=184
  StPassCmprtMdCtrl_Md24_VCUCfg_Val_write : Outport  Port=185
  StPassCmprtMdCtrl_Md25_VCUAvl_Val_write : Outport  Port=186
  StPassCmprtMdCtrl_Md25_VCUCfg_Val_write : Outport  Port=187
  StPassCmprtMdCtrl_Md26_VCUAvl_Val_write : Outport  Port=188
  StPassCmprtMdCtrl_Md26_VCUCfg_Val_write : Outport  Port=189
  StPassCmprtMdCtrl_Md27_VCUAvl_Val_write : Outport  Port=190
  StPassCmprtMdCtrl_Md27_VCUCfg_Val_write : Outport  Port=191
  StPassCmprtMdCtrl_Md28_VCUAvl_Val_write : Outport  Port=192
  StPassCmprtMdCtrl_Md28_VCUCfg_Val_write : Outport  Port=193
  StPassCmprtMdCtrl_Md29_VCUAvl_Val_write : Outport  Port=194
  StPassCmprtMdCtrl_Md29_VCUCfg_Val_write : Outport  Port=195
  StPassCmprtMdCtrl_Md3_VCUAvl_Val_write : Outport  Port=196
  StPassCmprtMdCtrl_Md3_VCUCfg_Val_write : Outport  Port=197
  StPassCmprtMdCtrl_Md30_VCUAvl_Val_write : Outport  Port=198
  StPassCmprtMdCtrl_Md30_VCUCfg_Val_write : Outport  Port=199
  StPassCmprtMdCtrl_Md31_VCUAvl_Val_write : Outport  Port=200
  StPassCmprtMdCtrl_Md31_VCUCfg_Val_write : Outport  Port=201
  StPassCmprtMdCtrl_Md32_VCUAvl_Val_write : Outport  Port=202
  StPassCmprtMdCtrl_Md32_VCUCfg_Val_write : Outport  Port=203
  StPassCmprtMdCtrl_Md4_VCUAvl_Val_write : Outport  Port=204
  StPassCmprtMdCtrl_Md4_VCUCfg_Val_write : Outport  Port=205
  StPassCmprtMdCtrl_Md5_VCUAvl_Val_write : Outport  Port=206
  StPassCmprtMdCtrl_Md5_VCUCfg_Val_write : Outport  Port=207
  StPassCmprtMdCtrl_Md6_VCUAvl_Val_write : Outport  Port=208
  StPassCmprtMdCtrl_Md6_VCUCfg_Val_write : Outport  Port=209
  StPassCmprtMdCtrl_Md7_VCUAvl_Val_write : Outport  Port=210
  StPassCmprtMdCtrl_Md7_VCUCfg_Val_write : Outport  Port=211
  StPassCmprtMdCtrl_Md8_VCUAvl_Val_write : Outport  Port=212
  StPassCmprtMdCtrl_Md8_VCUCfg_Val_write : Outport  Port=213
  StPassCmprtMdCtrl_Md9_VCUAvl_Val_write : Outport  Port=214
  StPassCmprtMdCtrl_Md9_VCUCfg_Val_write : Outport  Port=215
  StPassCmprtMdRfCtrlSwCstStAvl_Val_write : Outport  Port=216
  StSrvAvl_Md1_Val_write : Outport  Port=217
  StSrvAvl_Md10_Val_write : Outport  Port=218
  StSrvAvl_Md11_Val_write : Outport  Port=219
  StSrvAvl_Md13_Val_write : Outport  Port=220
  StSrvAvl_Md12_Val_write : Outport  Port=221
  StSrvAvl_Md14_Val_write : Outport  Port=222
  StSrvAvl_Md15_Val_write : Outport  Port=223
  StSrvAvl_Md16_Val_write : Outport  Port=224
  StSrvAvl_Md17_Val_write : Outport  Port=225
  StSrvAvl_Md18_Val_write : Outport  Port=226
  StSrvAvl_Md19_Val_write : Outport  Port=227
  StSrvAvl_Md2_Val_write : Outport  Port=228
  StSrvAvl_Md20_Val_write : Outport  Port=229
  StSrvAvl_Md21_Val_write : Outport  Port=230
  StSrvAvl_Md22_Val_write : Outport  Port=231
  StSrvAvl_Md23_Val_write : Outport  Port=232
  StSrvAvl_Md24_Val_write : Outport  Port=233
  StSrvAvl_Md25_Val_write : Outport  Port=234
  StSrvAvl_Md26_Val_write : Outport  Port=235
  StSrvAvl_Md27_Val_write : Outport  Port=236
  StSrvAvl_Md28_Val_write : Outport  Port=237
  StSrvAvl_Md29_Val_write : Outport  Port=238
  StSrvAvl_Md3_Val_write : Outport  Port=239
  StSrvAvl_Md30_Val_write : Outport  Port=240
  StSrvAvl_Md31_Val_write : Outport  Port=241
  StSrvAvl_Md32_Val_write : Outport  Port=242
  StSrvAvl_Md4_Val_write : Outport  Port=243
  StSrvAvl_Md5_Val_write : Outport  Port=244
  StSrvAvl_Md6_Val_write : Outport  Port=245
  StSrvAvl_Md7_Val_write : Outport  Port=246
  StSrvAvl_Md8_Val_write : Outport  Port=247
  StSrvAvl_Md9_Val_write : Outport  Port=248
  StSrvCfg_Md1_Val_write : Outport  Port=249
  StSrvCfg_Md10_Val_write : Outport  Port=250
  StSrvCfg_Md11_Val_write : Outport  Port=251
  StSrvCfg_Md12_Val_write : Outport  Port=252
  StSrvCfg_Md13_Val_write : Outport  Port=253
  StSrvCfg_Md14_Val_write : Outport  Port=254
  StSrvCfg_Md15_Val_write : Outport  Port=255
  StSrvCfg_Md16_Val_write : Outport  Port=256
  StSrvCfg_Md17_Val_write : Outport  Port=257
  StSrvCfg_Md18_Val_write : Outport  Port=258
  StSrvCfg_Md19_Val_write : Outport  Port=259
  StSrvCfg_Md2_Val_write : Outport  Port=260
  StSrvCfg_Md20_Val_write : Outport  Port=261
  StSrvCfg_Md21_Val_write : Outport  Port=262
  StSrvCfg_Md22_Val_write : Outport  Port=263
  StSrvCfg_Md23_Val_write : Outport  Port=264
  StSrvCfg_Md24_Val_write : Outport  Port=265
  StSrvCfg_Md25_Val_write : Outport  Port=266
  StSrvCfg_Md26_Val_write : Outport  Port=267
  StSrvCfg_Md27_Val_write : Outport  Port=268
  StSrvCfg_Md28_Val_write : Outport  Port=269
  StSrvCfg_Md29_Val_write : Outport  Port=270
  StSrvCfg_Md3_Val_write : Outport  Port=271
  StSrvCfg_Md30_Val_write : Outport  Port=272
  StSrvCfg_Md31_Val_write : Outport  Port=273
  StSrvCfg_Md32_Val_write : Outport  Port=274
  StSrvCfg_Md4_Val_write : Outport  Port=275
  StSrvCfg_Md5_Val_write : Outport  Port=276
  StSrvCfg_Md6_Val_write : Outport  Port=277
  StSrvCfg_Md7_Val_write : Outport  Port=278
  StSrvCfg_Md8_Val_write : Outport  Port=279
  StSrvCfg_Md9_Val_write : Outport  Port=280
  VipMdLtAvl_Val_write : Outport  Port=281
  VipMdRtAvl_Val_write : Outport  Port=282
  AcsEntry4s2LAvl_Val_write : Outport  Port=283
  AcsEntry4s2RAvl_Val_write : Outport  Port=284
  AcsEntryAll4sBwdAvl_Val_write : Outport  Port=285
  AcsEntryAll4sFwdAvl_Val_write : Outport  Port=286
  AcsExit4s2LAvl_Val_write : Outport  Port=287
  AcsExit4s2RAvl_Val_write : Outport  Port=288
  PasReclinerAvl_Val_write : Outport  Port=289
  unfold3LAvl_Val_write : Outport  Port=290
  unfold3RAvl_Val_write : Outport  Port=291
  VipLtOutMdAvl_Val_write : Outport  Port=292
  VipRtOutMdAvl_Val_write : Outport  Port=293
  PasReclinerExitAvl_Val_write : Outport  Port=294
  StPassCmprtMdCtrl_Md53_VCUAvl_Val_write : Outport  Port=295
  StPassCmprtMdCtrl_Md53_VCUCfg_Val_write : Outport  Port=296
  StPassCmprtMdCtrl_Md56_VCUAvl_Val_write : Outport  Port=297
  StPassCmprtMdCtrl_Md56_VCUCfg_Val_write : Outport  Port=298
  StPassCmprtMdCtrl_Md57_VCUAvl_Val_write : Outport  Port=299
  StPassCmprtMdCtrl_Md57_VCUCfg_Val_write : Outport  Port=300
  StPassCmprtMdCtrl_Md58_VCUAvl_Val_write : Outport  Port=301
  StPassCmprtMdCtrl_Md58_VCUCfg_Val_write : Outport  Port=302
  Big4SeatAvl_Val_write : Outport  Port=303
  StPassCmprtMdCtrl_Md61_VCUAvl_Val_write : Outport  Port=304
  StPassCmprtMdCtrl_Md62_VCUAvl_Val_write : Outport  Port=305
  M61WholeVehMemAvl_Val_write : Outport  Port=306
  M62WholeVehMemAvl_Val_write : Outport  Port=307
  StPassCmprtMdCtrl_Md61_VCUCfg_Val_write : Outport  Port=308
  StPassCmprtMdCtrl_Md62_VCUCfg_Val_write : Outport  Port=309
  wires:
  PA_HMI_2L_StMd12_Config_Val/1 -> Terminator_56/1
  PA_HMI_2L_StMd13_Config_Val/1 -> Terminator_57/1
  PA_HMI_2L_StMd15_Config_Val/1 -> Terminator_59/1
  PA_HMI_2L_StMd18_Config_Val/1 -> Terminator_62/1
  PA_HMI_2L_StMd19_Config_Val/1 -> Terminator_63/1
  PA_HMI_2L_StMd20_Config_Val/1 -> Terminator_65/1
  PA_HMI_2L_StMd23_Config_Val/1 -> Terminator_68/1
  PA_HMI_2L_StMd24_Config_Val/1 -> Terminator_69/1
  PA_HMI_2L_StMd27_Config_Val/1 -> Terminator_72/1
  PA_HMI_2L_StMd28_Config_Val/1 -> Terminator_73/1
  PA_HMI_2L_StMd29_Config_Val/1 -> Terminator_74/1
  PA_HMI_2L_StMd30_Config_Val/1 -> Terminator_76/1
  PA_HMI_2L_StMd31_Config_Val/1 -> Terminator_77/1
  PA_HMI_2L_StMd32_Config_Val/1 -> Terminator_78/1
  PA_HMI_2L_StMd6_Config_Val/1 -> Terminator_82/1
  PA_HMI_2L_StMd9_Config_Val/1 -> Terminator_85/1
  PA_HMI_2R_StMd10_Config_Val/1 -> Terminator_86/1
  PA_HMI_2R_StMd11_Config_Val/1 -> Terminator_87/1
  PA_HMI_2R_StMd14_Config_Val/1 -> Terminator_90/1
  PA_HMI_2R_StMd16_Config_Val/1 -> Terminator_92/1
  PA_HMI_2R_StMd17_Config_Val/1 -> Terminator_93/1
  PA_HMI_2R_StMd21_Config_Val/1 -> Terminator_98/1
  PA_HMI_2R_StMd22_Config_Val/1 -> Terminator_99/1
  PA_HMI_2R_StMd27_Config_Val/1 -> Terminator_104/1
  PA_HMI_2R_StMd28_Config_Val/1 -> Terminator_105/1
  PA_HMI_2R_StMd29_Config_Val/1 -> Terminator_106/1
  PA_HMI_2R_StMd30_Config_Val/1 -> Terminator_108/1
  PA_HMI_2R_StMd31_Config_Val/1 -> Terminator_109/1
  PA_HMI_2R_StMd32_Config_Val/1 -> Terminator_110/1
  PA_HMI_2R_StMd5_Config_Val/1 -> Terminator_113/1
  PA_HMI_2R_StMd7_Config_Val/1 -> Terminator_115/1
  PA_HMI_2R_StMd8_Config_Val/1 -> Terminator_116/1
  Ground_36/1 -> HMIMd16Avl_2R_Val_write/1
  Ground_40/1 -> HMIMd17Avl_2R_Val_write/1
  Ground_43/1 -> HMIMd18Avl_2L_Val_write/1
  Ground_47/1 -> HMIMd19Avl_2L_Val_write/1
  Ground_55/1 -> HMIMd20Avl_2L_Val_write/1
  Ground_57/1 -> HMIMd20Cfg_2L_Val_write/1
  Ground_60/1 -> HMIMd21Avl_2R_Val_write/1
  Ground_62/1 -> HMIMd21Cfg_2R_Val_write/1
  Ground_64/1 -> HMIMd22Avl_2R_Val_write/1
  Ground_66/1 -> HMIMd22Cfg_2R_Val_write/1
  Ground_67/1 -> HMIMd23Avl_2L_Val_write/1
  Ground_69/1 -> HMIMd23Cfg_2L_Val_write/1
  Ground_71/1 -> HMIMd24Avl_2L_Val_write/1
  Ground_73/1 -> HMIMd24Cfg_2L_Val_write/1
  Ground_83/1 -> HMIMd27Avl_2L_Val_write/1
  Ground_84/1 -> HMIMd27Avl_2R_Val_write/1
  Ground_85/1 -> HMIMd27Cfg_2L_Val_write/1
  Ground_86/1 -> HMIMd27Cfg_2R_Val_write/1
  Ground_87/1 -> HMIMd28Avl_2L_Val_write/1
  Ground_88/1 -> HMIMd28Avl_2R_Val_write/1
  Ground_89/1 -> HMIMd28Cfg_2L_Val_write/1
  Ground_90/1 -> HMIMd28Cfg_2R_Val_write/1
  Ground_91/1 -> HMIMd29Avl_2L_Val_write/1
  Ground_92/1 -> HMIMd29Avl_2R_Val_write/1
  Ground_93/1 -> HMIMd29Cfg_2L_Val_write/1
  Ground_94/1 -> HMIMd29Cfg_2R_Val_write/1
  Ground_99/1 -> HMIMd30Avl_2L_Val_write/1
  Ground_100/1 -> HMIMd30Avl_2R_Val_write/1
  Ground_101/1 -> HMIMd30Cfg_2L_Val_write/1
  Ground_102/1 -> HMIMd30Cfg_2R_Val_write/1
  Ground_103/1 -> HMIMd31Avl_2L_Val_write/1
  Ground_104/1 -> HMIMd31Avl_2R_Val_write/1
  Ground_105/1 -> HMIMd31Cfg_2L_Val_write/1
  Ground_106/1 -> HMIMd31Cfg_2R_Val_write/1
  Ground_107/1 -> HMIMd32Avl_2L_Val_write/1
  Ground_108/1 -> HMIMd32Avl_2R_Val_write/1
  Ground_109/1 -> HMIMd32Cfg_2L_Val_write/1
  Ground_110/1 -> HMIMd32Cfg_2R_Val_write/1
  Ground_120/1 -> HMIMd5Avl_2R_Val_write/1
  AbgDplyBckp_Val_read/1 -> Subsystem3/6(AbgDplyBckp)
  AbgDplyBckpV_Val_read/1 -> Subsystem3/7(AbgDplyBckpV)
  IsDrvStSwAct_Val_read/1 -> Subsystem3/30(IsDrvStSwAct)
  IsPasStSwAct_Val_read/1 -> Subsystem3/31(IsPasStSwAct)
  Is2LStSwAct_Val_read/1 -> Subsystem3/32(Is2LStSwAct)
  Is2RStSwAct_Val_read/1 -> Subsystem3/33(Is2RStSwAct)
  Is3LStSwAct_Val_read/1 -> Subsystem3/34(Is3LStSwAct)
  Is3RStSwAct_Val_read/1 -> Subsystem3/35(Is3RStSwAct)
  LugLtPosLrnd_Val_read/1 -> Subsystem3/21(LugLtPosLrnd)
  LugRtPosLrnd_Val_read/1 -> Subsystem3/22(LugRtPosLrnd)
  VIPLtPosLrnd_Val_read/1 -> Subsystem3/19(VIPLtPosLrnd)
  VIPRtPosLrnd_Val_read/1 -> Subsystem3/20(VIPRtPosLrnd)
  SysPwrMd_Val_read/1 -> Subsystem3/1(SysPwrMd)
  SysPwrMdV_Val_read/1 -> Subsystem3/2(SysPwrMdV)
  EnergyMgLdShdRq_Val_read/1 -> Subsystem3/4(EnergyMgLdShdRq)
  MmryRclImpctDisRq_Val_read/1 -> Subsystem3/5(MmryRclImpctDisRq)
  RcvyLtPosLrnd_Val_read/1 -> Subsystem3/23(RcvyLtPosLrnd)
  RcvyRtPosLrnd_Val_read/1 -> Subsystem3/24(RcvyRtPosLrnd)
  ThdRwLtStOccStatMSMSrc_Val_read/1 -> Subsystem3/25(ThdRwLtStOccStatMSMSrc)
  ThdRwCtStOccStatMSMSrc_Val_read/1 -> Subsystem3/26(ThdRwCtStOccStatMSMSrc)
  ThdRwRtStOccStatMSMSrc_Val_read/1 -> Subsystem3/27(ThdRwRtStOccStatMSMSrc)
  SecRwLtStChldLkReq_Val_read/1 -> Subsystem3/28(SecRwLtStChldLkReq)
  SecRwRtStChldLkReq_Val_read/1 -> Subsystem3/29(SecRwRtStChldLkReq)
  PassStPosRclRspStat_Val_read/1 -> Subsystem3/12(PassStPosRclRspStat)
  SecRwLtStPosRclRspStat_Val_read/1 -> Subsystem3/13(SecRwLtStPosRclRspStat)
  SecRwRtStPosRclRspStat_Val_read/1 -> Subsystem3/14(SecRwRtStPosRclRspStat)
  ThdRwLtStPosRclRspStat_Val_read/1 -> Subsystem3/15(ThdRwLtStPosRclRspStat)
  ThdRwRtStPosRclRspStat_Val_read/1 -> Subsystem3/16(ThdRwRtStPosRclRspStat)
  AcsExitPosLrnd_Val_read/1 -> Subsystem3/18(AcsExitPosLrnd)
  VoltSts_Val_read/1 -> Subsystem3/3(VoltSts)
  VehMovState_Val_read/1 -> Subsystem3/8(VehMovState)
  VehSpdAvgDrvn_Val_read/1 -> Subsystem3/10(VehSpdAvgDrvn)
  VehSpdAvgDrvnV_Val_read/1 -> Subsystem3/9(VehSpdAvgDrvnV)
  DrvStPosRclRspStat_Val_read/1 -> Subsystem3/11(DrvStPosRclRspStat)
  AcsEntryPosLrnd_Val_read/1 -> Subsystem3/17(AcsEntryPosLrnd)
  IntimacyLPosLrnd_Val_read/1 -> Subsystem3/44(IntimacyLPosLrnd)
  IntimacyRPosLrnd_Val_read/1 -> Subsystem3/45(IntimacyRPosLrnd)
  FamilyLtPosLrnd_Val_read/1 -> Subsystem3/46(FamilyLtPosLrnd)
  FamilyRtPosLrnd_Val_read/1 -> Subsystem3/47(FamilyRtPosLrnd)
  LyingLtPosLrnd_Val_read/1 -> Subsystem3/48(LyingLtPosLrnd)
  LyingRtPosLrnd_Val_read/1 -> Subsystem3/49(LyingRtPosLrnd)
  LgrstCloseLtPosLrnd_Val_read/1 -> Subsystem3/103(LgrstCloseLtPosLrnd)
  LgrstOpenLtPosLrnd_Val_read/1 -> Subsystem3/102(LgrstOpenLtPosLrnd)
  LgrstOpenRtPosLrnd_Val_read/1 -> Subsystem3/104(LgrstOpenRtPosLrnd)
  LgrstCloseRtPosLrnd_Val_read/1 -> Subsystem3/105(LgrstCloseRtPosLrnd)
  VeSignalLost2R_463_2L_Val_read/1 -> Subsystem3/36(VeSignalLost2R_463_2L)
  VeSignalLost3L_468_2L_Val_read/1 -> Subsystem3/37(VeSignalLost3L_468_2L)
  VeSignalLost3R_46C_2L_Val_read/1 -> Subsystem3/38("VeSignalLost3R_46C_2L ")
  VeSignalLostSDM_195_2L_Val_read/1 -> Subsystem3/42(VeSignalLostSDM_195_2L)
  VeSignalLostFireWall_1D2_2L_Val_read/1 -> Subsystem3/43(VeSignalLostFireWall_1D2_2L)
  VeSignalLostDR_213_2L_Val_read/1 -> Subsystem3/40(VeSignalLostDR_213_2L)
  VeSignalLostCODR_470_2L_Val_read/1 -> Subsystem3/39(VeSignalLostCODR_470_2L)
  PA_KeSMSbRoofSWEnable_Val/1 -> Subsystem3/41(KeSMSbRoofSWEnable)
  PA_StPassCmprtMdCtrl_Md14_VCUConfig_Val/1 -> Subsystem3/98(StPassCmprtMdCtrl_Md14_VCUConfig)
  PA_StPassCmprtMdCtrl_Md15_VCUConfig_Val/1 -> Subsystem3/99(StPassCmprtMdCtrl_Md15_VCUConfig)
  PA_StPassCmprtMdCtrl_Md7_VCUConfig_Val/1 -> Subsystem3/94(StPassCmprtMdCtrl_Md7_VCUConfig)
  PA_StPassCmprtMdCtrl_Md6_VCUConfig_Val/1 -> Subsystem3/92(StPassCmprtMdCtrl_Md6_VCUConfig)
  PA_StPassCmprtMdCtrl_Md5_VCUConfig_Val/1 -> Subsystem3/86(StPassCmprtMdCtrl_Md5_VCUConfig)
  PA_StPassCmprtMdCtrl_Md20_VCUConfig_Val/1 -> Subsystem3/87(StPassCmprtMdCtrl_Md20_VCUConfig)
  PA_StPassCmprtMdCtrl_Md13_VCUConfig_Val/1 -> Subsystem3/83(StPassCmprtMdCtrl_Md13_VCUConfig)
  PA_StPassCmprtMdCtrl_Md11_VCUConfig_Val/1 -> Subsystem3/82(StPassCmprtMdCtrl_Md11_VCUConfig)
  PA_StPassCmprtMdCtrl_Md9_VCUConfig_Val/1 -> Subsystem3/77(StPassCmprtMdCtrl_Md9_VCUConfig)
  PA_StPassCmprtMdCtrl_Md8_VCUConfig_Val/1 -> Subsystem3/75(StPassCmprtMdCtrl_Md8_VCUConfig)
  PA_StPassCmprtMdCtrl_Md3_VCUConfig_Val/1 -> Subsystem3/71(StPassCmprtMdCtrl_Md3_VCUConfig)
  PA_StPassCmprtMdCtrl_Md12_VCUConfig_Val/1 -> Subsystem3/63(StPassCmprtMdCtrl_Md12_VCUConfig)
  PA_StPassCmprtMdCtrl_Md19_VCUConfig_Val/1 -> Subsystem3/116(StPassCmprtMdCtrl_Md19_VCUConfig)
  PA_StPassCmprtMdCtrl_Md17_VCUConfig_Val/1 -> Subsystem3/110(StPassCmprtMdCtrl_Md17_VCUConfig)
  PA_StPassCmprtMdCtrl_Md18_VCUConfig_Val/1 -> Subsystem3/113(StPassCmprtMdCtrl_Md18_VCUConfig)
  PA_StPassCmprtMdCtrl_Md16_VCUConfig_Val/1 -> Subsystem3/107(StPassCmprtMdCtrl_Md16_VCUConfig)
  PA_StPassCmprtMdCtrl_Md4_VCUConfig_Val/1 -> Subsystem3/67(StPassCmprtMdCtrl_Md4_VCUConfig)
  PA_StPassCmprtMdCtrl_Md2_VCUConfig_Val/1 -> Subsystem3/56(StPassCmprtMdCtrl_Md2_VCUConfig)
  PA_StPassCmprtMdCtrl_Md1_VCUConfig_Val/1 -> Subsystem3/52(StPassCmprtMdCtrl_Md1_VCUConfig)
  PA_StPassCmprtMdCtrl_Md10_VCUConfig_Val/1 -> Subsystem3/62(StPassCmprtMdCtrl_Md10_VCUConfig)
  PA_HMI_2R_StMd12_Config_Val/1 -> Subsystem3/59(HMI_2R_StMd12_Config)
  PA_HMI_2L_StMd10_Config_Val/1 -> Subsystem3/58(HMI_2L_StMd10_Config)
  PA_HMI_2L_StMd2_Config_Val/1 -> Subsystem3/54(HMI_2L_StMd2_Config)
  PA_HMI_2R_StMd2_Config_Val/1 -> Subsystem3/55(HMI_2R_StMd2_Config)
  PA_HMI_2L_StMd1_Config_Val/1 -> Subsystem3/50(HMI_2L_StMd1_Config)
  PA_HMI_2R_StMd1_Config_Val/1 -> Subsystem3/51(HMI_2R_StMd1_Config)
  PA_HMI_2L_StMd4_Config_Val/1 -> Subsystem3/64(HMI_2L_StMd4_Config)
  PA_HMI_2R_StMd4_Config_Val/1 -> Subsystem3/65(HMI_2R_StMd4_Config)
  PA_HMI_2R_StMd3_Config_Val/1 -> Subsystem3/69(HMI_2R_StMd3_Config)
  PA_HMI_2L_StMd3_Config_Val/1 -> Subsystem3/68(HMI_2L_StMd3_Config)
  PA_HMI_2L_StMd8_Config_Val/1 -> Subsystem3/72(HMI_2L_StMd8_Config)
  PA_HMI_2R_StMd9_Config_Val/1 -> Subsystem3/73(HMI_2R_StMd9_Config)
  PA_HMI_2L_StMd11_Config_Val/1 -> Subsystem3/78(HMI_2L_StMd11_Config)
  PA_HMI_2R_StMd13_Config_Val/1 -> Subsystem3/79(HMI_2R_StMd13_Config)
  PA_HMI_2L_StMd5_Config_Val/1 -> Subsystem3/84(HMI_2L_StMd5_Config)
  PA_HMI_2R_StMd20_Config_Val/1 -> Subsystem3/85(HMI_2R_StMd20_Config)
  PA_HMI_2R_StMd6_Config_Val/1 -> Subsystem3/90(HMI_2R_StMd6_Config)
  PA_HMI_2L_StMd7_Config_Val/1 -> Subsystem3/91(HMI_2L_StMd7_Config)
  PA_HMI_2R_StMd15_Config_Val/1 -> Subsystem3/97(HMI_2R_StMd15_Config)
  PA_HMI_2L_StMd14_Config_Val/1 -> Subsystem3/96(HMI_2L_StMd14_Config)
  PA_HMI_2L_StMd16_Config_Val/1 -> Subsystem3/106(HMI_2L_StMd16_Config)
  PA_HMI_2L_StMd17_Config_Val/1 -> Subsystem3/109(HMI_2L_StMd17_Config)
  PA_HMI_2R_StMd19_Config_Val/1 -> Subsystem3/115(HMI_2R_StMd19_Config)
  PA_HMI_2R_StMd18_Config_Val/1 -> Subsystem3/112(HMI_2R_StMd18_Config)
  PA_StSrv_StMd19_Config_Val/1 -> Subsystem3/117(StSrv_StMd19_Config)
  PA_StSrv_StMd18_Config_Val/1 -> Subsystem3/114(StSrv_StMd18_Config)
  PA_StSrv_StMd17_Config_Val/1 -> Subsystem3/111(StSrv_StMd17_Config)
  PA_StSrv_StMd16_Config_Val/1 -> Subsystem3/108(StSrv_StMd16_Config)
  PA_StSrv_StMd15_Config_Val/1 -> Subsystem3/101(StSrv_StMd15_Config)
  PA_StSrv_StMd14_Config_Val/1 -> Subsystem3/100(StSrv_StMd14_Config)
  PA_StSrv_StMd6_Config_Val/1 -> Subsystem3/93(StSrv_StMd6_Config)
  PA_StSrv_StMd7_Config_Val/1 -> Subsystem3/95(StSrv_StMd7_Config)
  PA_StSrv_StMd5_Config_Val/1 -> Subsystem3/88(StSrv_StMd5_Config)
  PA_StSrv_StMd20_Config_Val/1 -> Subsystem3/89(StSrv_StMd20_Config)
  PA_StSrv_StMd11_Config_Val/1 -> Subsystem3/80(StSrv_StMd11_Config)
  PA_StSrv_StMd13_Config_Val/1 -> Subsystem3/81(StSrv_StMd13_Config)
  PA_StSrv_StMd9_Config_Val/1 -> Subsystem3/76(StSrv_StMd9_Config)
  PA_StSrv_StMd8_Config_Val/1 -> Subsystem3/74(StSrv_StMd8_Config)
  PA_StSrv_StMd3_Config_Val/1 -> Subsystem3/70(StSrv_StMd3_Config)
  PA_StSrv_StMd4_Config_Val/1 -> Subsystem3/66(StSrv_StMd4_Config)
  PA_StSrv_StMd10_Config_Val/1 -> Subsystem3/60(StSrv_StMd10_Config)
  PA_StSrv_StMd12_Config_Val/1 -> Subsystem3/61(StSrv_StMd12_Config)
  PA_StSrv_StMd2_Config_Val/1 -> Subsystem3/57(StSrv_StMd2_Config)
  PA_StSrv_StMd1_Config_Val/1 -> Subsystem3/53(StSrv_StMd1_Config)
  Subsystem3/1(CommCond) -> CommCond_Val_write/1
  Subsystem3/3(CommExitCond) -> CommExitCond_Val_write/1
  Subsystem3/2(CommExitCondwithSpeed) -> CommExitCondwithSpeed_Val_write/1
  Subsystem3/5(HMIMd1Cfg_2L) -> HMIMd1Cfg_2L_Val_write/1
  Subsystem3/6(HMIMd1Cfg_2R) -> HMIMd1Cfg_2R_Val_write/1
  Subsystem3/7(HMIMd1Avl_2L) -> HMIMd1Avl_2L_Val_write/1
  Subsystem3/8(HMIMd1Avl_2R) -> HMIMd1Avl_2R_Val_write/1
  Subsystem3/9(HMIMd2Cfg_2L) -> HMIMd2Cfg_2L_Val_write/1
  Subsystem3/10(HMIMd2Cfg_2R) -> HMIMd2Cfg_2R_Val_write/1
  Subsystem3/11(HMIMd2Avl_2L) -> HMIMd2Avl_2L_Val_write/1
  Subsystem3/12(HMIMd2Avl_2R) -> HMIMd2Avl_2R_Val_write/1
  Subsystem3/13(HMIMd3Cfg_2L) -> HMIMd3Cfg_2L_Val_write/1
  Subsystem3/14(HMIMd3Cfg_2R) -> HMIMd3Cfg_2R_Val_write/1
  Subsystem3/15(HMIMd3Avl_2L) -> HMIMd3Avl_2L_Val_write/1
  Subsystem3/16(HMIMd3Avl_2R) -> HMIMd3Avl_2R_Val_write/1
  Subsystem3/17(HMIMd4Cfg_2L) -> HMIMd4Cfg_2L_Val_write/1
  Subsystem3/18(HMIMd4Cfg_2R) -> HMIMd4Cfg_2R_Val_write/1
  Subsystem3/19(HMIMd4Avl_2L) -> HMIMd4Avl_2L_Val_write/1
  Subsystem3/20(HMIMd4Avl_2R) -> HMIMd4Avl_2R_Val_write/1
  Subsystem3/21(HMIMd6Cfg_2L) -> HMIMd6Cfg_2L_Val_write/1
  Subsystem3/22(HMIMd6Avl_2L) -> HMIMd6Avl_2L_Val_write/1
  Subsystem3/23(HMIMd7Cfg_2R) -> HMIMd7Cfg_2R_Val_write/1
  Subsystem3/24(HMIMd7Avl_2R) -> HMIMd7Avl_2R_Val_write/1
  Subsystem3/26(HMIMd8Cfg_2R) -> HMIMd8Cfg_2R_Val_write/1
  Subsystem3/25(HMIMd8Cfg_2L) -> HMIMd8Cfg_2L_Val_write/1
  Subsystem3/27(HMIMd8Avl_2L) -> HMIMd8Avl_2L_Val_write/1
  Subsystem3/28(HMIMd8Avl_2R) -> HMIMd8Avl_2R_Val_write/1
  Subsystem3/29(HMIMd9Cfg_2L) -> HMIMd9Cfg_2L_Val_write/1
  Subsystem3/30(HMIMd9Cfg_2R) -> HMIMd9Cfg_2R_Val_write/1
  Subsystem3/31(HMIMd9Avl_2L) -> HMIMd9Avl_2L_Val_write/1
  Subsystem3/32(HMIMd9Avl_2R) -> HMIMd9Avl_2R_Val_write/1
  Subsystem3/4(PwrMdChked) -> PwrMdChked_Val_write/1
  Subsystem3/108(IntimacyLMdAvl) -> IntimacyLMdAvl_Val_write/1
  Subsystem3/109(IntimacyRMdAvl) -> IntimacyRMdAvl_Val_write/1
  Subsystem3/106(RcvyMdLtAvl) -> RcvyMdLtAvl_Val_write/1
  Subsystem3/107(RcvyMdRtAvl) -> RcvyMdRtAvl_Val_write/1
  Subsystem3/104(LugMdLtAvl) -> LugMdLtAvl_Val_write/1
  Subsystem3/105(LugMdRtAvl) -> LugMdRtAvl_Val_write/1
  Subsystem3/113(LyingMdRtAvl) -> LyingMdRtAvl_Val_write/1
  Subsystem3/112(LyingMdLtAvl) -> LyingMdLtAvl_Val_write/1
  Subsystem3/103(VipMdRtAvl) -> VipMdRtAvl_Val_write/1
  Subsystem3/102("VipMdLtAvl ") -> VipMdLtAvl_Val_write/1
  Subsystem3/100(AcsMdEntyAvl) -> AcsMdEntyAvl_Val_write/1
  Subsystem3/101(AcsMdExtAvl) -> AcsMdExtAvl_Val_write/1
  Subsystem3/110(FamilyMdLtAvl) -> FamilyMdLtAvl_Val_write/1
  Subsystem3/111(FamilyMdRtAvl) -> FamilyMdRtAvl_Val_write/1
  Subsystem3/178(StPassCmprtMdCtrl_Md20_VCUAvl) -> StPassCmprtMdCtrl_Md20_VCUAvl_Val_write/1
  Subsystem3/152(StPassCmprtMdCtrl_Md16_VCUAvl) -> StPassCmprtMdCtrl_Md16_VCUAvl_Val_write/1
  Subsystem3/176(StPassCmprtMdCtrl_Md19_VCUAvl) -> StPassCmprtMdCtrl_Md19_VCUAvl_Val_write/1
  Subsystem3/141(StPassCmprtMdCtrl_Md15_VCUAvl) -> StPassCmprtMdCtrl_Md15_VCUAvl_Val_write/1
  Subsystem3/118(StPassCmprtMdCtrl_Md20_VCUCfg) -> StPassCmprtMdCtrl_Md20_VCUCfg_Val_write/1
  Subsystem3/117(StPassCmprtMdCtrl_Md5_VCUCfg) -> StPassCmprtMdCtrl_Md5_VCUCfg_Val_write/1
  Subsystem3/135(StPassCmprtMdCtrl_Md7_VCUAvl) -> StPassCmprtMdCtrl_Md7_VCUAvl_Val_write/1
  Subsystem3/132(StPassCmprtMdCtrl_Md6_VCUAvl) -> StPassCmprtMdCtrl_Md6_VCUAvl_Val_write/1
  Subsystem3/123(StPassCmprtMdCtrl_Md6_VCUCfg) -> StPassCmprtMdCtrl_Md6_VCUCfg_Val_write/1
  Subsystem3/124(StPassCmprtMdCtrl_Md7_VCUCfg) -> StPassCmprtMdCtrl_Md7_VCUCfg_Val_write/1
  Subsystem3/149(StPassCmprtMdCtrl_Md16_VCUCfg) -> StPassCmprtMdCtrl_Md16_VCUCfg_Val_write/1
  Subsystem3/156(StPassCmprtMdCtrl_Md17_VCUCfg) -> StPassCmprtMdCtrl_Md17_VCUCfg_Val_write/1
  Subsystem3/160(StPassCmprtMdCtrl_Md17_VCUAvl) -> StPassCmprtMdCtrl_Md17_VCUAvl_Val_write/1
  Subsystem3/165(StPassCmprtMdCtrl_Md18_VCUCfg) -> StPassCmprtMdCtrl_Md18_VCUCfg_Val_write/1
  Subsystem3/168(StPassCmprtMdCtrl_Md19_VCUCfg) -> StPassCmprtMdCtrl_Md19_VCUCfg_Val_write/1
  Subsystem3/129(StPassCmprtMdCtrl_Md5_VCUAvl) -> StPassCmprtMdCtrl_Md5_VCUAvl_Val_write/1
  Subsystem3/138(StPassCmprtMdCtrl_Md14_VCUAvl) -> StPassCmprtMdCtrl_Md14_VCUAvl_Val_write/1
  Subsystem3/146(LgrstOpenLtMdAvl) -> LgrstOpenLtMdAvl_Val_write/1
  Subsystem3/158(LgrstCloseLtMdAvl) -> LgrstCloseLtMdAvl_Val_write/1
  Subsystem3/170(LgrstOpenRtMdAvl) -> LgrstOpenRtMdAvl_Val_write/1
  Subsystem3/174(LgrstCloseRtMdAvl) -> LgrstCloseRtMdAvl_Val_write/1
  Subsystem3/143(DiagAbgDly) -> DiagAbgDly_Val_write/1
  Subsystem3/144(DiagVehMovState) -> DiagVehMovState_Val_write/1
  Subsystem3/145(DiagVehSpdAvgDrvn) -> DiagVehSpdAvgDrvn_Val_write/1
  Subsystem3/99(StPassCmprtMdRfCtrlSwCstStAvl) -> StPassCmprtMdRfCtrlSwCstStAvl_Val_write/1
  Subsystem3/172(StPassCmprtMdCtrl_Md18_VCUAvl) -> StPassCmprtMdCtrl_Md18_VCUAvl_Val_write/1
  Subsystem3/55(StPassCmprtMdCtrl_Md1_VCUAvl) -> StPassCmprtMdCtrl_Md1_VCUAvl_Val_write/1
  Subsystem3/65(StPassCmprtMdCtrl_Md1_VCUCfg) -> StPassCmprtMdCtrl_Md1_VCUCfg_Val_write/1
  Subsystem3/61(StPassCmprtMdCtrl_Md10_VCUAvl) -> StPassCmprtMdCtrl_Md10_VCUAvl_Val_write/1
  Subsystem3/62(StPassCmprtMdCtrl_Md11_VCUAvl) -> StPassCmprtMdCtrl_Md11_VCUAvl_Val_write/1
  Subsystem3/63(StPassCmprtMdCtrl_Md12_VCUAvl) -> StPassCmprtMdCtrl_Md12_VCUAvl_Val_write/1
  Subsystem3/64(StPassCmprtMdCtrl_Md13_VCUAvl) -> StPassCmprtMdCtrl_Md13_VCUAvl_Val_write/1
  Subsystem3/74(StPassCmprtMdCtrl_Md13_VCUCfg) -> StPassCmprtMdCtrl_Md13_VCUCfg_Val_write/1
  Subsystem3/73(StPassCmprtMdCtrl_Md12_VCUCfg) -> StPassCmprtMdCtrl_Md12_VCUCfg_Val_write/1
  Subsystem3/72(StPassCmprtMdCtrl_Md11_VCUCfg) -> StPassCmprtMdCtrl_Md11_VCUCfg_Val_write/1
  Subsystem3/71(StPassCmprtMdCtrl_Md10_VCUCfg) -> StPassCmprtMdCtrl_Md10_VCUCfg_Val_write/1
  Subsystem3/66(StPassCmprtMdCtrl_Md2_VCUCfg) -> StPassCmprtMdCtrl_Md2_VCUCfg_Val_write/1
  Subsystem3/67(StPassCmprtMdCtrl_Md3_VCUCfg) -> StPassCmprtMdCtrl_Md3_VCUCfg_Val_write/1
  Subsystem3/56(StPassCmprtMdCtrl_Md2_VCUAvl) -> StPassCmprtMdCtrl_Md2_VCUAvl_Val_write/1
  Subsystem3/57(StPassCmprtMdCtrl_Md3_VCUAvl) -> StPassCmprtMdCtrl_Md3_VCUAvl_Val_write/1
  Subsystem3/58(StPassCmprtMdCtrl_Md4_VCUAvl) -> StPassCmprtMdCtrl_Md4_VCUAvl_Val_write/1
  Subsystem3/59(StPassCmprtMdCtrl_Md8_VCUAvl) -> StPassCmprtMdCtrl_Md8_VCUAvl_Val_write/1
  Subsystem3/60(StPassCmprtMdCtrl_Md9_VCUAvl) -> StPassCmprtMdCtrl_Md9_VCUAvl_Val_write/1
  Subsystem3/68(StPassCmprtMdCtrl_Md4_VCUCfg) -> StPassCmprtMdCtrl_Md4_VCUCfg_Val_write/1
  Subsystem3/69(StPassCmprtMdCtrl_Md8_VCUCfg) -> StPassCmprtMdCtrl_Md8_VCUCfg_Val_write/1
  Subsystem3/70(StPassCmprtMdCtrl_Md9_VCUCfg) -> StPassCmprtMdCtrl_Md9_VCUCfg_Val_write/1
  Subsystem3/75(StPassCmprtMdCtrl_Md14_VCUCfg) -> StPassCmprtMdCtrl_Md14_VCUCfg_Val_write/1
  Subsystem3/76(StPassCmprtMdCtrl_Md15_VCUCfg) -> StPassCmprtMdCtrl_Md15_VCUCfg_Val_write/1
  Subsystem3/179(StSrvAvl_Md20) -> StSrvAvl_Md20_Val_write/1
  Subsystem3/177(StSrvAvl_Md19) -> StSrvAvl_Md19_Val_write/1
  Subsystem3/173(StSrvAvl_Md18) -> StSrvAvl_Md18_Val_write/1
  Subsystem3/161(StSrvAvl_Md17) -> StSrvAvl_Md17_Val_write/1
  Subsystem3/153(StSrvAvl_Md16) -> StSrvAvl_Md16_Val_write/1
  Subsystem3/139(StSrvAvl_Md14) -> StSrvAvl_Md14_Val_write/1
  Subsystem3/142(StSrvAvl_Md15) -> StSrvAvl_Md15_Val_write/1
  Subsystem3/130(StSrvAvl_Md5) -> StSrvAvl_Md5_Val_write/1
  Subsystem3/133(StSrvAvl_Md6) -> StSrvAvl_Md6_Val_write/1
  Subsystem3/136(StSrvAvl_Md7) -> StSrvAvl_Md7_Val_write/1
  Subsystem3/98(StSrvAvl_Md13) -> StSrvAvl_Md13_Val_write/1
  Subsystem3/97(StSrvAvl_Md12) -> StSrvAvl_Md12_Val_write/1
  Subsystem3/96(StSrvAvl_Md11) -> StSrvAvl_Md11_Val_write/1
  Subsystem3/95(StSrvAvl_Md10) -> StSrvAvl_Md10_Val_write/1
  Subsystem3/94(StSrvAvl_Md9) -> StSrvAvl_Md9_Val_write/1
  Subsystem3/93(StSrvAvl_Md8) -> StSrvAvl_Md8_Val_write/1
  Subsystem3/92(StSrvAvl_Md4) -> StSrvAvl_Md4_Val_write/1
  Subsystem3/91(StSrvAvl_Md3) -> StSrvAvl_Md3_Val_write/1
  Subsystem3/90(StSrvAvl_Md2) -> StSrvAvl_Md2_Val_write/1
  Subsystem3/89(StSrvAvl_Md1) -> StSrvAvl_Md1_Val_write/1
  Subsystem3/166(StSrvCfg_Md18) -> StSrvCfg_Md18_Val_write/1
  Subsystem3/169(StSrvCfg_Md19) -> StSrvCfg_Md19_Val_write/1
  Subsystem3/157(StSrvCfg_Md17) -> StSrvCfg_Md17_Val_write/1
  Subsystem3/150(StSrvCfg_Md16) -> StSrvCfg_Md16_Val_write/1
  Subsystem3/125(StSrvCfg_Md6) -> StSrvCfg_Md6_Val_write/1
  Subsystem3/126(StSrvCfg_Md7) -> StSrvCfg_Md7_Val_write/1
  Subsystem3/120(StSrvCfg_Md20) -> StSrvCfg_Md20_Val_write/1
  Subsystem3/119(StSrvCfg_Md5) -> StSrvCfg_Md5_Val_write/1
  Subsystem3/77(StSrvCfg_Md1) -> StSrvCfg_Md1_Val_write/1
  Subsystem3/78(StSrvCfg_Md2) -> StSrvCfg_Md2_Val_write/1
  Subsystem3/79(StSrvCfg_Md3) -> StSrvCfg_Md3_Val_write/1
  Subsystem3/80(StSrvCfg_Md4) -> StSrvCfg_Md4_Val_write/1
  Subsystem3/81(StSrvCfg_Md8) -> StSrvCfg_Md8_Val_write/1
  Subsystem3/82(StSrvCfg_Md9) -> StSrvCfg_Md9_Val_write/1
  Subsystem3/83(StSrvCfg_Md10) -> StSrvCfg_Md10_Val_write/1
  Subsystem3/84(StSrvCfg_Md11) -> StSrvCfg_Md11_Val_write/1
  Subsystem3/85(StSrvCfg_Md12) -> StSrvCfg_Md12_Val_write/1
  Subsystem3/86(StSrvCfg_Md13) -> StSrvCfg_Md13_Val_write/1
  Subsystem3/87(StSrvCfg_Md14) -> StSrvCfg_Md14_Val_write/1
  Subsystem3/88(StSrvCfg_Md15) -> StSrvCfg_Md15_Val_write/1
  Subsystem3/33(HMIMd10Cfg_2L) -> HMIMd10Cfg_2L_Val_write/1
  Subsystem3/34(HMIMd10Cfg_2R) -> HMIMd10Cfg_2R_Val_write/1
  Subsystem3/35(HMIMd10Avl_2L) -> HMIMd10Avl_2L_Val_write/1
  Subsystem3/36(HMIMd10Avl_2R) -> HMIMd10Avl_2R_Val_write/1
  Subsystem3/37(HMIMd11Cfg_2L) -> HMIMd11Cfg_2L_Val_write/1
  Subsystem3/38(HMIMd11Cfg_2R) -> HMIMd11Cfg_2R_Val_write/1
  Subsystem3/39(HMIMd11Avl_2L) -> HMIMd11Avl_2L_Val_write/1
  Subsystem3/40(HMIMd11Avl_2R) -> HMIMd11Avl_2R_Val_write/1
  Subsystem3/41(HMIMd12Cfg_2L) -> HMIMd12Cfg_2L_Val_write/1
  Subsystem3/42(HMIMd12Cfg_2R) -> HMIMd12Cfg_2R_Val_write/1
  Subsystem3/43(HMIMd12Avl_2L) -> HMIMd12Avl_2L_Val_write/1
  Subsystem3/44(HMIMd12Avl_2R) -> HMIMd12Avl_2R_Val_write/1
  Subsystem3/45(HMIMd13Cfg_2L) -> HMIMd13Cfg_2L_Val_write/1
  Subsystem3/46(HMIMd13Cfg_2R) -> HMIMd13Cfg_2R_Val_write/1
  Subsystem3/47(HMIMd13Avl_2L) -> HMIMd13Avl_2L_Val_write/1
  Subsystem3/48(HMIMd13Avl_2R) -> HMIMd13Avl_2R_Val_write/1
  Subsystem3/49(HMIMd14Cfg_2L) -> HMIMd14Cfg_2L_Val_write/1
  Subsystem3/50(HMIMd14Cfg_2R) -> HMIMd14Cfg_2R_Val_write/1
  Subsystem3/51(HMIMd14Avl_2R) -> HMIMd14Avl_2R_Val_write/1
  Subsystem3/52(HMIMd15Cfg_2L) -> HMIMd15Cfg_2L_Val_write/1
  Subsystem3/53(HMIMd15Cfg_2R) -> HMIMd15Cfg_2R_Val_write/1
  Subsystem3/54(HMIMd15Avl_2L) -> HMIMd15Avl_2L_Val_write/1
  Subsystem3/114(HMIMd5Cfg_2L) -> HMIMd5Cfg_2L_Val_write/1
  Subsystem3/115(HMIMd20Cfg_2R) -> HMIMd20Cfg_2R_Val_write/1
  Subsystem3/116(HMIMd5Cfg_2R) -> HMIMd5Cfg_2R_Val_write/1
  Subsystem3/128(HMIMd20Avl_2R) -> HMIMd20Avl_2R_Val_write/1
  Subsystem3/121(HMIMd6Cfg_2R) -> HMIMd6Cfg_2R_Val_write/1
  Subsystem3/122(HMIMd7Cfg_2L) -> HMIMd7Cfg_2L_Val_write/1
  Subsystem3/127(HMIMd5Avl_2L) -> HMIMd5Avl_2L_Val_write/1
  Subsystem3/131(HMIMd6Avl_2R) -> HMIMd6Avl_2R_Val_write/1
  Subsystem3/134(HMIMd7Avl_2L) -> HMIMd7Avl_2L_Val_write/1
  Subsystem3/137(HMIMd14Avl_2L) -> HMIMd14Avl_2L_Val_write/1
  Subsystem3/140(HMIMd15Avl_2R) -> HMIMd15Avl_2R_Val_write/1
  Subsystem3/148(HMIMd16Cfg_2R) -> HMIMd16Cfg_2R_Val_write/1
  Subsystem3/147(HMIMd16Cfg_2L) -> HMIMd16Cfg_2L_Val_write/1
  Subsystem3/151(HMIMd16Avl_2L) -> HMIMd16Avl_2L_Val_write/1
  Subsystem3/159(HMIMd17Avl_2L) -> HMIMd17Avl_2L_Val_write/1
  Subsystem3/162(HMIMd18Cfg_2L) -> HMIMd18Cfg_2L_Val_write/1
  Subsystem3/163(HMIMd19Cfg_2L) -> HMIMd19Cfg_2L_Val_write/1
  Subsystem3/164(HMIMd18Cfg_2R) -> HMIMd18Cfg_2R_Val_write/1
  Subsystem3/167(HMIMd19Cfg_2R) -> HMIMd19Cfg_2R_Val_write/1
  Subsystem3/171(HMIMd18Avl_2R) -> HMIMd18Avl_2R_Val_write/1
  Subsystem3/175(HMIMd19Avl_2R) -> HMIMd19Avl_2R_Val_write/1
  Subsystem3/154(HMIMd17Cfg_2R) -> HMIMd17Cfg_2R_Val_write/1
  Subsystem3/155(HMIMd17Cfg_2L) -> HMIMd17Cfg_2L_Val_write/1
  IfVeSMSeStNumConfig_Val_read/1 -> Subsystem3/118(IfVeSMSeStNumConfig)
  PA_KeSMSLegrstDisFwdBkwdPos_Val/1 -> Subsystem3/119(KeSMSLegrstDisFwdBkwdPos)
  SecRwLtStFrwdBkwdPos_Val_read/1 -> Subsystem3/120(SecRwLtStFrwdBkwdPos)
  SecRwLtStFrwdBkwdPosV_Val_read/1 -> Subsystem3/121("SecRwLtStFrwdBkwdPosV ")
  SecRwRtStFrwdBkwdPos_Val_read/1 -> Subsystem3/122("SecRwRtStFrwdBkwdPos ")
  SecRwRtStFrwdBkwdPosV_Val_read/1 -> Subsystem3/123("SecRwRtStFrwdBkwdPosV ")
  AcsEntry4s2LPosLrnd_Val_read/1 -> Subsystem3/124(AcsEntry4s2LPosLrnd)
  Subsystem3/180(AcsEntry4s2LAvl) -> AcsEntry4s2LAvl_Val_write/1
  PA_HMI_2L_StMd21_Config_Val/1 -> Subsystem3/125(HMI_2L_StMd21_Config)
  PA_StPassCmprtMdCtrl_Md21_VCUConfig_Val/1 -> Subsystem3/126(StPassCmprtMdCtrl_Md21_VCUConfig)
  PA_StSrv_StMd21_Config_Val/1 -> Subsystem3/127(StSrv_StMd21_Config)
  AcsEntry4s2RPosLrnd_Val_read/1 -> Subsystem3/128(AcsEntry4s2RPosLrnd)
  AcsExit4s2LPosLrnd_Val_read/1 -> Subsystem3/132(AcsExit4s2LPosLrnd)
  AcsExit4s2RPosLrnd_Val_read/1 -> Subsystem3/136(AcsExit4s2RPosLrnd)
  AcsEntryAll4sFwdPosLrnd_Val_read/1 -> Subsystem3/140(AcsEntryAll4sFwdPosLrnd)
  AcsEntryAll4sBwdPosLrnd_Val_read/1 -> Subsystem3/145(AcsEntryAll4sBwdPosLrnd)
  PA_HMI_2R_StMd23_Config_Val/1 -> Subsystem3/129(HMI_2R_StMd23_Config)
  PA_StPassCmprtMdCtrl_Md23_VCUConfig_Val/1 -> Subsystem3/130(StPassCmprtMdCtrl_Md23_VCUConfig)
  PA_StSrv_StMd23_Config_Val/1 -> Subsystem3/131(StSrv_StMd23_Config)
  PA_HMI_2L_StMd22_Config_Val/1 -> Subsystem3/133(HMI_2L_StMd22_Config)
  PA_StPassCmprtMdCtrl_Md22_VCUConfig_Val/1 -> Subsystem3/134(StPassCmprtMdCtrl_Md22_VCUConfig)
  PA_StSrv_StMd22_Config_Val/1 -> Subsystem3/135(StSrv_StMd22_Config)
  PA_HMI_2R_StMd24_Config_Val/1 -> Subsystem3/137(HMI_2R_StMd24_Config)
  PA_StPassCmprtMdCtrl_Md24_VCUConfig_Val/1 -> Subsystem3/138(StPassCmprtMdCtrl_Md24_VCUConfig)
  PA_StSrv_StMd24_Config_Val/1 -> Subsystem3/139(StSrv_StMd24_Config)
  PA_HMI_2L_StMd26_Config_Val/1 -> Subsystem3/141(HMI_2L_StMd26_Config)
  PA_HMI_2R_StMd26_Config_Val/1 -> Subsystem3/142(HMI_2R_StMd26_Config)
  PA_StPassCmprtMdCtrl_Md26_VCUConfig_Val/1 -> Subsystem3/143(StPassCmprtMdCtrl_Md26_VCUConfig)
  PA_StSrv_StMd26_Config_Val/1 -> Subsystem3/144(StSrv_StMd26_Config)
  PA_HMI_2L_StMd25_Config_Val/1 -> Subsystem3/146(HMI_2L_StMd25_Config)
  PA_HMI_2R_StMd25_Config_Val/1 -> Subsystem3/147(HMI_2R_StMd25_Config)
  PA_StPassCmprtMdCtrl_Md25_VCUConfig_Val/1 -> Subsystem3/148(StPassCmprtMdCtrl_Md25_VCUConfig)
  PA_StSrv_StMd25_Config_Val/1 -> Subsystem3/149(StSrv_StMd25_Config)
  Subsystem3/184(HMIMd21Cfg_2L) -> HMIMd21Cfg_2L_Val_write/1
  Subsystem3/181(HMIMd21Avl_2L) -> HMIMd21Avl_2L_Val_write/1
  Subsystem3/182(StPassCmprtMdCtrl_Md21_VCUAvl) -> StPassCmprtMdCtrl_Md21_VCUAvl_Val_write/1
  Subsystem3/185(StPassCmprtMdCtrl_Md21_VCUCfg) -> StPassCmprtMdCtrl_Md21_VCUCfg_Val_write/1
  Subsystem3/191(StPassCmprtMdCtrl_Md23_VCUAvl) -> StPassCmprtMdCtrl_Md23_VCUAvl_Val_write/1
  Subsystem3/189(StPassCmprtMdCtrl_Md23_VCUCfg) -> StPassCmprtMdCtrl_Md23_VCUCfg_Val_write/1
  Subsystem3/198(StPassCmprtMdCtrl_Md22_VCUAvl) -> StPassCmprtMdCtrl_Md22_VCUAvl_Val_write/1
  Subsystem3/196(StPassCmprtMdCtrl_Md22_VCUCfg) -> StPassCmprtMdCtrl_Md22_VCUCfg_Val_write/1
  Subsystem3/205(StPassCmprtMdCtrl_Md24_VCUAvl) -> StPassCmprtMdCtrl_Md24_VCUAvl_Val_write/1
  Subsystem3/203(StPassCmprtMdCtrl_Md24_VCUCfg) -> StPassCmprtMdCtrl_Md24_VCUCfg_Val_write/1
  Subsystem3/211(StPassCmprtMdCtrl_Md26_VCUCfg) -> StPassCmprtMdCtrl_Md26_VCUCfg_Val_write/1
  Subsystem3/215(StPassCmprtMdCtrl_Md26_VCUAvl) -> StPassCmprtMdCtrl_Md26_VCUAvl_Val_write/1
  Subsystem3/224(StPassCmprtMdCtrl_Md25_VCUAvl) -> StPassCmprtMdCtrl_Md25_VCUAvl_Val_write/1
  Subsystem3/220(StPassCmprtMdCtrl_Md25_VCUCfg) -> StPassCmprtMdCtrl_Md25_VCUCfg_Val_write/1
  Subsystem3/217(AcsEntryAll4sBwdAvl) -> AcsEntryAll4sBwdAvl_Val_write/1
  Subsystem3/208(AcsEntryAll4sFwdAvl) -> AcsEntryAll4sFwdAvl_Val_write/1
  Subsystem3/201(AcsExit4s2RAvl) -> AcsExit4s2RAvl_Val_write/1
  Subsystem3/194(AcsExit4s2LAvl) -> AcsExit4s2LAvl_Val_write/1
  Subsystem3/187(AcsEntry4s2RAvl) -> AcsEntry4s2RAvl_Val_write/1
  Subsystem3/225(StSrvAvl_Md25) -> StSrvAvl_Md25_Val_write/1
  Subsystem3/221(StSrvCfg_Md25) -> StSrvCfg_Md25_Val_write/1
  Subsystem3/212(StSrvCfg_Md26) -> StSrvCfg_Md26_Val_write/1
  Subsystem3/216(StSrvAvl_Md26) -> StSrvAvl_Md26_Val_write/1
  Subsystem3/207(StSrvAvl_Md24) -> StSrvAvl_Md24_Val_write/1
  Subsystem3/204(StSrvCfg_Md24) -> StSrvCfg_Md24_Val_write/1
  Subsystem3/193(StSrvAvl_Md23) -> StSrvAvl_Md23_Val_write/1
  Subsystem3/190(StSrvCfg_Md23) -> StSrvCfg_Md23_Val_write/1
  Subsystem3/200(StSrvAvl_Md22) -> StSrvAvl_Md22_Val_write/1
  Subsystem3/197(StSrvCfg_Md22) -> StSrvCfg_Md22_Val_write/1
  Subsystem3/183(StSrvAvl_Md21) -> StSrvAvl_Md21_Val_write/1
  Subsystem3/186(StSrvCfg_Md21) -> StSrvCfg_Md21_Val_write/1
  Subsystem3/188(HMIMd23Cfg_2R) -> HMIMd23Cfg_2R_Val_write/1
  Subsystem3/192(HMIMd23Avl_2R) -> HMIMd23Avl_2R_Val_write/1
  Subsystem3/195(HMIMd22Cfg_2L) -> HMIMd22Cfg_2L_Val_write/1
  Subsystem3/199(HMIMd22Avl_2L) -> HMIMd22Avl_2L_Val_write/1
  Subsystem3/202(HMIMd24Cfg_2R) -> HMIMd24Cfg_2R_Val_write/1
  Subsystem3/206(HMIMd24Avl_2R) -> HMIMd24Avl_2R_Val_write/1
  Subsystem3/209(HMIMd26Cfg_2L) -> HMIMd26Cfg_2L_Val_write/1
  Subsystem3/210(HMIMd26Cfg_2R) -> HMIMd26Cfg_2R_Val_write/1
  Subsystem3/213(HMIMd26Avl_2L) -> HMIMd26Avl_2L_Val_write/1
  Subsystem3/214(HMIMd26Avl_2R) -> HMIMd26Avl_2R_Val_write/1
  Subsystem3/218(HMIMd25Cfg_2L) -> HMIMd25Cfg_2L_Val_write/1
  Subsystem3/219(HMIMd25Cfg_2R) -> HMIMd25Cfg_2R_Val_write/1
  Subsystem3/222(HMIMd25Avl_2L) -> HMIMd25Avl_2L_Val_write/1
  Subsystem3/223(HMIMd25Avl_2R) -> HMIMd25Avl_2R_Val_write/1
  PA_IfKeSMSbSeatMovFrwdBkwdEnable_Val/1 -> Subsystem3/150(IfKeSMSbSeatMovFrwdBkwdEnable)
  IfVeSMSbPassReclinerPosLrnd_Val_read/1 -> Subsystem3/151(PassReclinerPosLrnd)
  IfVeSMSbunfold3LPosLrnd_Val_read/1 -> Subsystem3/152(unfold3LPosLrnd)
  IfVeSMSbunfold3RPosLrnd_Val_read/1 -> Subsystem3/153(unfold3RPosLrnd)
  NotCoDrvStOccStatBDFSrc_Val_read/1 -> Subsystem3/154(NotCoDrvStOccStatBDFSrc)
  PA_StPassCmprtMdCtrl_Md30_VCUConfig_Val/1 -> Subsystem3/155(StPassCmprtMdCtrl_Md30_VCUConfig)
  PA_StPassCmprtMdCtrl_Md31_VCUConfig_Val/1 -> Subsystem3/157(StPassCmprtMdCtrl_Md31_VCUConfig)
  PA_StSrv_StMd30_Config_Val/1 -> Subsystem3/156(StSrv_StMd30_Config)
  PA_StSrv_StMd31_Config_Val/1 -> Subsystem3/158(StSrv_StMd31_Config)
  PA_StPassCmprtMdCtrl_Md32_VCUConfig_Val/1 -> Subsystem3/159(StPassCmprtMdCtrl_Md32_VCUConfig)
  PA_StSrv_StMd32_Config_Val/1 -> Subsystem3/160(StSrv_StMd32_Config)
  IfVeSMSbVIPLtOutPosLrnd_Val_read/1 -> Subsystem3/161(VIPLtOutPosLrnd)
  IfVeSMSbVIPRtOutPosLrnd_Val_read/1 -> Subsystem3/162(VIPRtOutPosLrnd)
  PA_StPassCmprtMdCtrl_Md27_VCUConfig_Val/1 -> Subsystem3/163(StPassCmprtMdCtrl_Md27_VCUConfig)
  PA_StPassCmprtMdCtrl_Md28_VCUConfig_Val/1 -> Subsystem3/165(StPassCmprtMdCtrl_Md28_VCUConfig)
  PA_StPassCmprtMdCtrl_Md29_VCUConfig_Val/1 -> Subsystem3/167(StPassCmprtMdCtrl_Md29_VCUConfig)
  PA_StSrv_StMd27_Config_Val/1 -> Subsystem3/164(StSrv_StMd27_Config)
  PA_StSrv_StMd28_Config_Val/1 -> Subsystem3/166(StSrv_StMd28_Config)
  PA_StSrv_StMd29_Config_Val/1 -> Subsystem3/168(StSrv_StMd29_Config)
  Subsystem3/227(StPassCmprtMdCtrl_Md30_VCUCfg) -> StPassCmprtMdCtrl_Md30_VCUCfg_Val_write/1
  Subsystem3/229(StPassCmprtMdCtrl_Md31_VCUCfg) -> StPassCmprtMdCtrl_Md31_VCUCfg_Val_write/1
  Subsystem3/231(StPassCmprtMdCtrl_Md30_VCUAvl) -> StPassCmprtMdCtrl_Md30_VCUAvl_Val_write/1
  Subsystem3/233(StPassCmprtMdCtrl_Md31_VCUAvl) -> StPassCmprtMdCtrl_Md31_VCUAvl_Val_write/1
  Subsystem3/236(StPassCmprtMdCtrl_Md32_VCUCfg) -> StPassCmprtMdCtrl_Md32_VCUCfg_Val_write/1
  Subsystem3/238(StPassCmprtMdCtrl_Md32_VCUAvl) -> StPassCmprtMdCtrl_Md32_VCUAvl_Val_write/1
  Subsystem3/243(StPassCmprtMdCtrl_Md29_VCUAvl) -> StPassCmprtMdCtrl_Md29_VCUAvl_Val_write/1
  Subsystem3/244(StPassCmprtMdCtrl_Md27_VCUAvl) -> StPassCmprtMdCtrl_Md27_VCUAvl_Val_write/1
  Subsystem3/245(StPassCmprtMdCtrl_Md28_VCUAvl) -> StPassCmprtMdCtrl_Md28_VCUAvl_Val_write/1
  Subsystem3/249(StPassCmprtMdCtrl_Md27_VCUCfg) -> StPassCmprtMdCtrl_Md27_VCUCfg_Val_write/1
  Subsystem3/251(StPassCmprtMdCtrl_Md28_VCUCfg) -> StPassCmprtMdCtrl_Md28_VCUCfg_Val_write/1
  Subsystem3/253(StPassCmprtMdCtrl_Md29_VCUCfg) -> StPassCmprtMdCtrl_Md29_VCUCfg_Val_write/1
  Subsystem3/228(StSrvCfg_Md30) -> StSrvCfg_Md30_Val_write/1
  Subsystem3/230(StSrvCfg_Md31) -> StSrvCfg_Md31_Val_write/1
  Subsystem3/232(StSrvAvl_Md30) -> StSrvAvl_Md30_Val_write/1
  Subsystem3/234(StSrvAvl_Md31) -> StSrvAvl_Md31_Val_write/1
  Subsystem3/237(StSrvCfg_Md32) -> StSrvCfg_Md32_Val_write/1
  Subsystem3/239(StSrvAvl_Md32) -> StSrvAvl_Md32_Val_write/1
  Subsystem3/247(StSrvAvl_Md27) -> StSrvAvl_Md27_Val_write/1
  Subsystem3/246(StSrvAvl_Md29) -> StSrvAvl_Md29_Val_write/1
  Subsystem3/248(StSrvAvl_Md28) -> StSrvAvl_Md28_Val_write/1
  Subsystem3/250(StSrvCfg_Md27) -> StSrvCfg_Md27_Val_write/1
  Subsystem3/254(StSrvCfg_Md29) -> StSrvCfg_Md29_Val_write/1
  Subsystem3/252(StSrvCfg_Md28) -> StSrvCfg_Md28_Val_write/1
  IfVeSMSuThdRwLtStCshnFldUpwdDnwdPos_Val_read/1 -> Subsystem3/169(ThdRwLtStCshnFldUpwdDnwdPos)
  IfVeSMSuThdRwLtStCshnFldUpwdDnwdPosV_Val_read/1 -> Subsystem3/170(ThdRwLtStCshnFldUpwdDnwdPosV)
  IfVeSMSuThdRwRtStCshnFldUpwdDnwdPos_Val_read/1 -> Subsystem3/171(ThdRwRtStCshnFldUpwdDnwdPos)
  IfVeSMSuThdRwRtStCshnFldUpwdDnwdPosV_Val_read/1 -> Subsystem3/172(ThdRwRtStCshnFldUpwdDnwdPosV)
  Subsystem3/226("PasReclinerAvl ") -> PasReclinerAvl_Val_write/1
  Subsystem3/235(unfold3LAvl) -> unfold3LAvl_Val_write/1
  Subsystem3/240(unfold3RAvl) -> unfold3RAvl_Val_write/1
  Subsystem3/241(VipLtOutMdAvl) -> VipLtOutMdAvl_Val_write/1
  Subsystem3/242(VipRtOutMdAvl) -> VipRtOutMdAvl_Val_write/1
  ThdRwLtStChldLkReq_Val_read/1 -> Subsystem3/173(ThdRwLtStChldLkReq)
  NotSecRowLeStOccStatBDFSrc_Val_read/1 -> Subsystem3/174(NotSecRowLeStOccStatBDFSrc)
  NotSecRowRtStOccStatBDFSrc_Val_read/1 -> Subsystem3/175(NotSecRowRtStOccStatBDFSrc)
  Subsystem3/255(PasReclinerExitAvl) -> PasReclinerExitAvl_Val_write/1
  IfVeSMSuSecRwLtStBkReclnUpwdDnwdPos_Val_read/1 -> Subsystem3/176(SecRwLtStBkReclnUpwdDnwdPos)
  IfVeSMSbSecRwLtStBkReclnUpwdDnwdPosV_Val_read/1 -> Subsystem3/177(SecRwLtStBkReclnUpwdDnwdPosV)
  IfVeSMSuSecRwRtStBkReclnUpwdDnwdPos_Val_read/1 -> Subsystem3/178(SecRwRtStBkReclnUpwdDnwdPos)
  IfVeSMSbSecRwRtStBkReclnUpwdDnwdPosV_Val_read/1 -> Subsystem3/179(SecRwRtStBkReclnUpwdDnwdPosV)
  PA_KeSMSuSecRwStBackPosDelta_Val/1 -> Subsystem3/180(KeSMSuSecRwStBackPosDelta)
  PA_StPassCmprtMdCtrl_Md53_VCUConfig_Val/1 -> Subsystem3/181(StPassCmprtMdCtrl_Md53_VCUConfig)
  Subsystem3/257(StPassCmprtMdCtrl_Md53_VCUAvl) -> StPassCmprtMdCtrl_Md53_VCUAvl_Val_write/1
  Subsystem3/256(StPassCmprtMdCtrl_Md53_VCUCfg) -> StPassCmprtMdCtrl_Md53_VCUCfg_Val_write/1
  PA_StPassCmprtMdCtrl_Md56_VCUConfig_Val/1 -> Subsystem3/182(StPassCmprtMdCtrl_Md56_VCUConfig)
  Subsystem3/258(StPassCmprtMdCtrl_Md56_VCUCfg) -> StPassCmprtMdCtrl_Md56_VCUCfg_Val_write/1
  Subsystem3/259(StPassCmprtMdCtrl_Md56_VCUAvl) -> StPassCmprtMdCtrl_Md56_VCUAvl_Val_write/1
  PA_StPassCmprtMdCtrl_Md57_VCUConfig_Val/1 -> Subsystem3/184(StPassCmprtMdCtrl_Md57_VCUConfig)
  PA_StPassCmprtMdCtrl_Md58_VCUConfig_Val/1 -> Subsystem3/185(StPassCmprtMdCtrl_Md58_VCUConfig)
  Subsystem3/260(StPassCmprtMdCtrl_Md57_VCUCfg) -> StPassCmprtMdCtrl_Md57_VCUCfg_Val_write/1
  Subsystem3/261(StPassCmprtMdCtrl_Md58_VCUCfg) -> StPassCmprtMdCtrl_Md58_VCUCfg_Val_write/1
  Subsystem3/262(StPassCmprtMdCtrl_Md57_VCUAvl) -> StPassCmprtMdCtrl_Md57_VCUAvl_Val_write/1
  Subsystem3/263(StPassCmprtMdCtrl_Md58_VCUAvl) -> StPassCmprtMdCtrl_Md58_VCUAvl_Val_write/1
  IfVeSMSbPasReclinerPosAvail_Val_read/1 -> Subsystem3/186(PasReclinerPosAvail)
  Subsystem3/264(Big4SeatAvl) -> Big4SeatAvl_Val_write/1
  PA_KeSMSuThrdRwCushFoldPosThreshold_Val/1 -> Subsystem3/183(KeSMSuThrdRwCushFoldPosThreshold)
  PA_KeSMSwAcsMd32SecRwLtStBkReclnUpwdDnwdPos1_Val/1 -> Subsystem3/187(KeSMSwAcsMd32SecRwLtStBkReclnUpwdDnwdPos1)
  PA_KeSMSwAcsMd53SecRwRtStBkReclnUpwdDnwdPos1_Val/1 -> Subsystem3/188(KeSMSwAcsMd53SecRwRtStBkReclnUpwdDnwdPos1)
  PA_KeSMSwAcsMd8SecRwLtStBkReclnUpwdDnwdPos_Val/1 -> Subsystem3/189(KeSMSwAcsMd8SecRwLtStBkReclnUpwdDnwdPos)
  PA_KeSMSwAcsMd9SecRwRtStBkReclnUpwdDnwdPos_Val/1 -> Subsystem3/190(KeSMSwAcsMd9SecRwRtStBkReclnUpwdDnwdPos)
  WholeVehMemPosLrnd_Val_read/1 -> Subsystem3/191(WholeVehMemPosLrnd)
  PA_StPassCmprtMdCtrl_Md61_VCUConfig_Val/1 -> Subsystem3/192(StPassCmprtMdCtrl_Md61_VCUConfig)
  PA_StPassCmprtMdCtrl_Md62_VCUConfig_Val/1 -> Subsystem3/193(StPassCmprtMdCtrl_Md62_VCUConfig)
  PA_KeSMSwSeatBkLimitPos_Val/1 -> Subsystem3/194(KeSMSwSeatBkLimitPos)
  PA_KeSMSwSeatBkLimitPosDelt_Val/1 -> Subsystem3/195(KeSMSwSeatBkLimitPosDelt)
  Md61PassStBkReclnTrgtPos_Val_read/1 -> Subsystem3/196(Md61PassStBkReclnTrgtPos)
  Md61ThdRwLtStCshnFldUpwdDnwdTrgtPos_Val_read/1 -> Subsystem3/197(Md61ThdRwLtStCshnFldUpwdDnwdTrgtPos)
  Md61ThdRwRtStCshnFldUpwdDnwdTrgtPos_Val_read/1 -> Subsystem3/198(Md61ThdRwRtStCshnFldUpwdDnwdTrgtPos)
  Md62PassStBkReclnTrgtPos_Val_read/1 -> Subsystem3/199(Md62PassStBkReclnTrgtPos)
  Md62ThdRwLtStCshnFldUpwdDnwdTrgtPos_Val_read/1 -> Subsystem3/200(Md62ThdRwLtStCshnFldUpwdDnwdTrgtPos)
  Md62ThdRwRtStCshnFldUpwdDnwdTrgtPos_Val_read/1 -> Subsystem3/201(Md62ThdRwRtStCshnFldUpwdDnwdTrgtPos)
  PA_KeSMSuThrdRwCushFoldPosDelta_Val/1 -> Subsystem3/202(KeSMSuThrdRwCushFoldPosDelta)
  Subsystem3/265(StPassCmprtMdCtrl_Md61_VCUAvl) -> StPassCmprtMdCtrl_Md61_VCUAvl_Val_write/1
  Subsystem3/266(StPassCmprtMdCtrl_Md62_VCUAvl) -> StPassCmprtMdCtrl_Md62_VCUAvl_Val_write/1
  Subsystem3/267(M61WholeVehMemAvl) -> M61WholeVehMemAvl_Val_write/1
  Subsystem3/268(M62WholeVehMemAvl) -> M62WholeVehMemAvl_Val_write/1
  Subsystem3/269(StPassCmprtMdCtrl_Md61_VCUCfg) -> StPassCmprtMdCtrl_Md61_VCUCfg_Val_write/1
  Subsystem3/270(StPassCmprtMdCtrl_Md62_VCUCfg) -> StPassCmprtMdCtrl_Md62_VCUCfg_Val_write/1
